simulink model "Parallel_n49"  (R2012b)
settings: Solver=VariableStepDiscrete  StartTime=0.0  StopTime=TotalIterations  RelTol=1e-3
values from neighbouring files (symbols this model uses):
  bp = 12    [ConfigValidate.m]
  bpSNMemory = bp    (= 12)    [ConfigValidate.m]
  IterationsOrdering = 4000    [ConfigValidate.m]
  MaxCoordDistance = (abs(max(wx) - min(wx))+abs(max(wy) - min(wy)))^2    [ConfigValidate.m]
  N_limit = 0.01    [ConfigValidate.m]
  nBits = 9    [ConfigValidate.m]
  nBitsNSmemories = (ceil(log2(TotalIterations)))    [ConfigValidate.m]
  S_limit = 1    [ConfigValidate.m]
  SourceNodes = 2000    [ConfigValidate.m]
  ts = 1    [ConfigValidate.m]
  w1 = rand(1,Neurons)    [ConfigValidate.m]
  w2 = rand(1,Neurons)    [ConfigValidate.m]
  wx = zeros(1,Neurons)    [ConfigValidate.m]
  wy = zeros(1,Neurons)    [ConfigValidate.m]
  x1 = rand(SourceNodes,1)    [ConfigValidate.m]
  x2 = rand(SourceNodes,1)    [ConfigValidate.m]
libraries: xbsIndex_r4 x4147, dspsrcs4 x2, dspstat3 x2
(part 3 of 19)

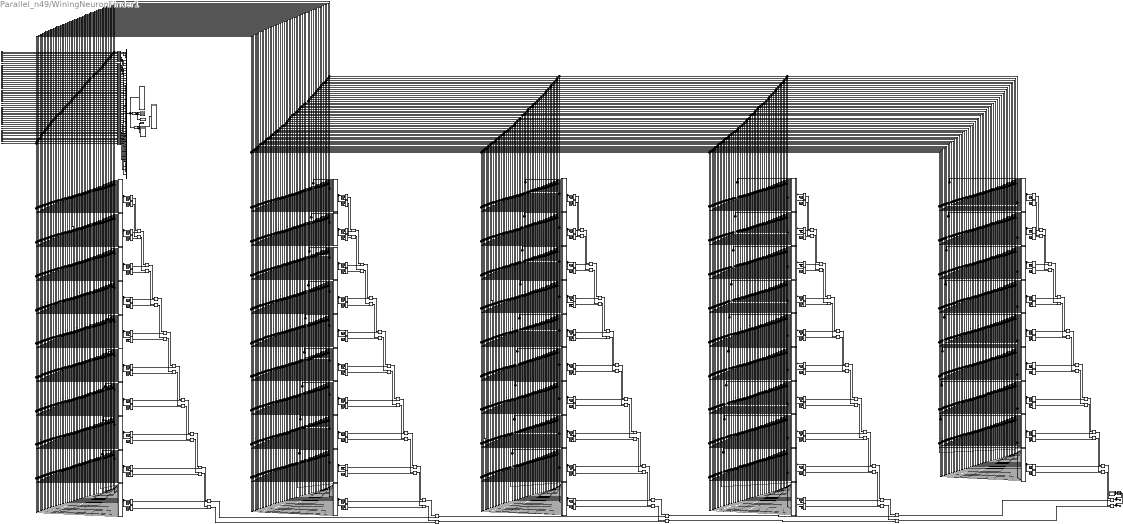
== system Parallel_n49/WiningNeuronFinder1 ==
  dist_k1 : Inport
  dist_k2 : Inport  Port=2
  dist_k3 : Inport  Port=3
  dist_k4 : Inport  Port=4
  dist_k5 : Inport  Port=5
  dist_k6 : Inport  Port=6
  dist_k7 : Inport  Port=7
  dist_k8 : Inport  Port=8
  dist_k9 : Inport  Port=9
  dist_k10 : Inport  Port=10
  dist_k11 : Inport  Port=11
  dist_k12 : Inport  Port=12
  dist_k13 : Inport  Port=13
  dist_k14 : Inport  Port=14
  dist_k15 : Inport  Port=15
  dist_k16 : Inport  Port=16
  dist_k17 : Inport  Port=17
  dist_k18 : Inport  Port=18
  dist_k19 : Inport  Port=19
  dist_k20 : Inport  Port=20
  dist_k21 : Inport  Port=21
  dist_k22 : Inport  Port=22
  dist_k23 : Inport  Port=23
  dist_k24 : Inport  Port=24
  dist_k25 : Inport  Port=25
  dist_k26 : Inport  Port=26
  dist_k27 : Inport  Port=27
  dist_k28 : Inport  Port=28
  dist_k29 : Inport  Port=29
  dist_k30 : Inport  Port=30
  dist_k31 : Inport  Port=31
  dist_k32 : Inport  Port=32
  dist_k33 : Inport  Port=33
  dist_k34 : Inport  Port=34
  dist_k35 : Inport  Port=35
  dist_k36 : Inport  Port=36
  dist_k37 : Inport  Port=37
  dist_k38 : Inport  Port=38
  dist_k39 : Inport  Port=39
  dist_k40 : Inport  Port=40
  dist_k41 : Inport  Port=41
  dist_k42 : Inport  Port=42
  dist_k43 : Inport  Port=43
  dist_k44 : Inport  Port=44
  dist_k45 : Inport  Port=45
  dist_k46 : Inport  Port=46
  dist_k47 : Inport  Port=47
  dist_k48 : Inport  Port=48
  dist_k49 : Inport  Port=49
  wx_1 : Inport  Port=50
  wy_1 : Inport  Port=51
  wx_2 : Inport  Port=52
  wy_2 : Inport  Port=53
  wx_3 : Inport  Port=54
  wy_3 : Inport  Port=55
  wx_4 : Inport  Port=56
  wy_4 : Inport  Port=57
  wx_5 : Inport  Port=58
  wy_5 : Inport  Port=59
  wx_6 : Inport  Port=60
  wy_6 : Inport  Port=61
  wx_7 : Inport  Port=62
  wy_7 : Inport  Port=63
  wx_8 : Inport  Port=64
  wy_8 : Inport  Port=65
  wx_9 : Inport  Port=66
  wy_9 : Inport  Port=67
  wx_10 : Inport  Port=68
  wy_10 : Inport  Port=69
  wx_11 : Inport  Port=70
  wy_11 : Inport  Port=71
  wx_12 : Inport  Port=72
  wy_12 : Inport  Port=73
  wx_13 : Inport  Port=74
  wy_13 : Inport  Port=75
  wx_14 : Inport  Port=76
  wy_14 : Inport  Port=77
  wx_15 : Inport  Port=78
  wy_15 : Inport  Port=79
  wx_16 : Inport  Port=80
  wy_16 : Inport  Port=81
  wx_17 : Inport  Port=82
  wy_17 : Inport  Port=83
  wx_18 : Inport  Port=84
  wy_18 : Inport  Port=85
  wx_19 : Inport  Port=86
  wy_19 : Inport  Port=87
  wx_20 : Inport  Port=88
  wy_20 : Inport  Port=89
  wx_21 : Inport  Port=90
  wy_21 : Inport  Port=91
  wx_22 : Inport  Port=92
  wy_22 : Inport  Port=93
  wx_23 : Inport  Port=94
  wy_23 : Inport  Port=95
  wx_24 : Inport  Port=96
  wy_24 : Inport  Port=97
  wx_25 : Inport  Port=98
  wy_25 : Inport  Port=99
  wx_26 : Inport  Port=100
  wy_26 : Inport  Port=101
  wx_27 : Inport  Port=102
  wy_27 : Inport  Port=103
  wx_28 : Inport  Port=104
  wy_28 : Inport  Port=105
  wx_29 : Inport  Port=106
  wy_29 : Inport  Port=107
  wx_30 : Inport  Port=108
  wy_30 : Inport  Port=109
  wx_31 : Inport  Port=110
  wy_31 : Inport  Port=111
  wx_32 : Inport  Port=112
  wy_32 : Inport  Port=113
  wx_33 : Inport  Port=114
  wy_33 : Inport  Port=115
  wx_34 : Inport  Port=116
  wy_34 : Inport  Port=117
  wx_35 : Inport  Port=118
  wy_35 : Inport  Port=119
  wx_36 : Inport  Port=120
  wy_36 : Inport  Port=121
  wx_37 : Inport  Port=122
  wy_37 : Inport  Port=123
  wx_38 : Inport  Port=124
  wy_38 : Inport  Port=125
  wx_39 : Inport  Port=126
  wy_39 : Inport  Port=127
  wx_40 : Inport  Port=128
  wy_40 : Inport  Port=129
  wx_41 : Inport  Port=130
  wy_41 : Inport  Port=131
  wx_42 : Inport  Port=132
  wy_42 : Inport  Port=133
  wx_43 : Inport  Port=134
  wy_43 : Inport  Port=135
  wx_44 : Inport  Port=136
  wy_44 : Inport  Port=137
  wx_45 : Inport  Port=138
  wy_45 : Inport  Port=139
  wx_46 : Inport  Port=140
  wy_46 : Inport  Port=141
  wx_47 : Inport  Port=142
  wy_47 : Inport  Port=143
  wx_48 : Inport  Port=144
  wy_48 : Inport  Port=145
  wx_49 : Inport  Port=146
  wy_49 : Inport  Port=147
  Display{,1..3,54..55} (6 alike) : Display
  Gateway Out{,1..28,31..42,44..53} (51 alike) : xbsIndex_r4/Gateway Out  inherit_from_input=off  hdl_port=off  timing_constraint=None  locs_specified=off  LOCs={}  UseAsDAC=off  DACChannel='1'  block_type=gatewayout
  LowerDist_n1 : Subsystem
  LowerDist_n10 : Subsystem
  LowerDist_n11 : Subsystem
  LowerDist_n12 : Subsystem
  LowerDist_n13 : Subsystem
  LowerDist_n14 : Subsystem
  LowerDist_n15 : Subsystem
  LowerDist_n16 : Subsystem
  LowerDist_n17 : Subsystem
  LowerDist_n18 : Subsystem
  LowerDist_n19 : Subsystem
  LowerDist_n2 : Subsystem
  LowerDist_n20 : Subsystem
  LowerDist_n21 : Subsystem
  LowerDist_n22 : Subsystem
  LowerDist_n23 : Subsystem
  LowerDist_n24 : Subsystem
  LowerDist_n25 : Subsystem
  LowerDist_n26 : Subsystem
  LowerDist_n27 : Subsystem
  LowerDist_n28 : Subsystem
  LowerDist_n29 : Subsystem
  LowerDist_n3 : Subsystem
  LowerDist_n30 : Subsystem
  LowerDist_n31 : Subsystem
  LowerDist_n32 : Subsystem
  LowerDist_n33 : Subsystem
  LowerDist_n34 : Subsystem
  LowerDist_n35 : Subsystem
  LowerDist_n36 : Subsystem
  LowerDist_n37 : Subsystem
  LowerDist_n38 : Subsystem
  LowerDist_n39 : Subsystem
  LowerDist_n4 : Subsystem
  LowerDist_n40 : Subsystem
  LowerDist_n41 : Subsystem
  LowerDist_n42 : Subsystem
  LowerDist_n43 : Subsystem
  LowerDist_n44 : Subsystem
  LowerDist_n45 : Subsystem
  LowerDist_n46 : Subsystem
  LowerDist_n47 : Subsystem
  LowerDist_n48 : Subsystem
  LowerDist_n49 : Subsystem
  LowerDist_n5 : Subsystem
  LowerDist_n6 : Subsystem
  LowerDist_n7 : Subsystem
  LowerDist_n8 : Subsystem
  LowerDist_n9 : Subsystem
  Minimum : dspstat3/Minimum  fcn=Value and Index  reset=None  InputProcessing=Columns as channels (frame based)  indexBase=One  operateOver=Each column  Dimension=1  colComp=on  operation=minimum  roiEnable=off  roiType=Rectangles  roiPortion=Entire ROI  roiOutput=Individual statistics for each ROI  roiFlag=off  roundingMode=Floor  overflowMode=off
  Mux : Mux  Inputs=49
  Mux2 : Mux  Inputs=2
  Sort : dspstat3/Sort  otype=Value and Index  dir=Ascending  sortAlg=Quick sort  accumDataTypeStr=Inherit: Same as product output  accumLastDataTypeStr=Inherit: Same as product output  roundingMode=Floor  overflowMode=off
  Sum_wxWinning_n{1..96} (96 alike) : xbsIndex_r4/AddSub  mode=Addition  use_carryin=off  use_carryout=off  en=off  latency=dAdd_CooperatingProcess  precision=User Defined  arith_type=Unsigned  n_bits=nbCoord  bin_pt=bpCoord  quantization=Truncate  overflow=Wrap  dbl_ovrd=off  use_behavioral_HDL=off  hw_selection=Fabric  pipelined=off  block_type=addsub
  To Workspace : ToWorkspace  VariableName=win_histH  SampleTime=ts
  To Workspace1 : ToWorkspace  VariableName=win_distH  SampleTime=ts
  wy_doMenor{,1..89,92..99} (98 alike) : xbsIndex_r4/Mux  inputs=2  en=off  latency=dMUX_CompetitiveProcess  precision=Full  arith_type=Unsigned  n_bits=16  bin_pt=14  quantization=Truncate  overflow=Wrap  dbl_ovrd=off  block_type=mux
  zero{,1..89,92..99} (98 alike) : xbsIndex_r4/Constant  const=0  gui_display_data_type=Fixed-point  arith_type=Unsigned  n_bits=nbCoord  bin_pt=bpCoord  preci_type=Single  exp_width=8  frac_width=24  explicit_period=on  period=ts  equ=P=C  opselect=C  inp2=PCIN>>17  opr=+  inp1=P  carry=CIN  dbl_ovrd=off  block_type=constant
  WinningNeuron_wx : Outport
  WinningNeuron_wy : Outport  Port=2
  wires:
  wy_1/1 -> wy_doMenor1/3
  wx_1/1 -> wy_doMenor/3
  Gateway Out6/1 -> Mux/7
  Gateway Out5/1 -> Mux/6
  Gateway Out7/1 -> Mux/8
  Gateway Out4/1 -> Mux/5
  Gateway Out8/1 -> Mux/9
  Gateway Out1/1 -> Mux/2
  Gateway Out3/1 -> Mux/4
  Gateway Out2/1 -> Mux/3
  Gateway Out10/1 -> Mux/11
  Gateway Out11/1 -> Mux/12
  Gateway Out9/1 -> Mux/10
  Gateway Out/1 -> Mux/1
  Gateway Out12/1 -> Mux/13
  Gateway Out22/1 -> Mux/17
  Gateway Out13/1 -> Mux/14
  Gateway Out14/1 -> Mux/15
  Gateway Out15/1 -> Mux/16
  Gateway Out23/1 -> Mux/18
  Gateway Out16/1 -> Mux/20
  Gateway Out17/1 -> Mux/21
  Gateway Out24/1 -> Mux/19
  Gateway Out18/1 -> Mux/22
  Gateway Out20/1 -> Mux/24
  Gateway Out21/1 -> Mux/25
  Gateway Out19/1 -> Mux/23
  LowerDist_n1/1(Out1) -> wy_doMenor1/1, wy_doMenor/1
  zero/1 -> wy_doMenor/2
  zero1/1 -> wy_doMenor1/2
  wy_doMenor/1 -> Sum_wxWinning_n1/1
  wy_doMenor1/1 -> Sum_wxWinning_n2/1
  Gateway Out25/1 -> Mux/26
  Gateway Out26/1 -> Mux/27
  Gateway Out41/1 -> Mux/28
  Gateway Out47/1 -> Mux/29
  Gateway Out48/1 -> Mux/30
  Gateway Out49/1 -> Mux/31
  Gateway Out51/1 -> Mux/33
  Gateway Out50/1 -> Mux/32
  Gateway Out52/1 -> Mux/34
  Gateway Out31/1 -> Mux/36
  Gateway Out32/1 -> Mux/37
  Gateway Out53/1 -> Mux/35
  Gateway Out33/1 -> Mux/38
  Gateway Out34/1 -> Mux/39
  Gateway Out35/1 -> Mux/40
  Gateway Out36/1 -> Mux/41
  Gateway Out44/1 -> Mux/42
  Gateway Out45/1 -> Mux/43
  Gateway Out38/1 -> Mux/46
  Gateway Out37/1 -> Mux/45
  Gateway Out46/1 -> Mux/44
  Gateway Out39/1 -> Mux/47
  Gateway Out42/1 -> Mux/49
  Gateway Out40/1 -> Mux/48
  wy_2/1 -> wy_doMenor3/3
  wx_2/1 -> wy_doMenor2/3
  LowerDist_n2/1(Out1) -> wy_doMenor3/1, wy_doMenor2/1
  zero2/1 -> wy_doMenor2/2
  zero3/1 -> wy_doMenor3/2
  wy_3/1 -> wy_doMenor5/3
  wx_3/1 -> wy_doMenor4/3
  LowerDist_n3/1(Out1) -> wy_doMenor5/1, wy_doMenor4/1
  zero4/1 -> wy_doMenor4/2
  zero5/1 -> wy_doMenor5/2
  wy_4/1 -> wy_doMenor7/3
  wx_4/1 -> wy_doMenor6/3
  LowerDist_n4/1(Out1) -> wy_doMenor7/1, wy_doMenor6/1
  zero6/1 -> wy_doMenor6/2
  zero7/1 -> wy_doMenor7/2
  wy_5/1 -> wy_doMenor9/3
  wx_5/1 -> wy_doMenor8/3
  LowerDist_n5/1(Out1) -> wy_doMenor9/1, wy_doMenor8/1
  zero8/1 -> wy_doMenor8/2
  zero9/1 -> wy_doMenor9/2
  wy_6/1 -> wy_doMenor11/3
  wx_6/1 -> wy_doMenor10/3
  LowerDist_n6/1(Out1) -> wy_doMenor11/1, wy_doMenor10/1
  zero10/1 -> wy_doMenor10/2
  zero11/1 -> wy_doMenor11/2
  wy_7/1 -> wy_doMenor13/3
  wx_7/1 -> wy_doMenor12/3
  LowerDist_n7/1(Out1) -> wy_doMenor13/1, wy_doMenor12/1
  zero12/1 -> wy_doMenor12/2
  zero13/1 -> wy_doMenor13/2
  wy_8/1 -> wy_doMenor15/3
  wx_8/1 -> wy_doMenor14/3
  LowerDist_n8/1(Out1) -> wy_doMenor15/1, wy_doMenor14/1
  zero14/1 -> wy_doMenor14/2
  zero15/1 -> wy_doMenor15/2
  wy_9/1 -> wy_doMenor17/3
  wx_9/1 -> wy_doMenor16/3
  LowerDist_n9/1(Out1) -> wy_doMenor17/1, wy_doMenor16/1
  zero16/1 -> wy_doMenor16/2
  zero17/1 -> wy_doMenor17/2
  wy_10/1 -> wy_doMenor19/3
  wx_10/1 -> wy_doMenor18/3
  LowerDist_n10/1(Out1) -> wy_doMenor19/1, wy_doMenor18/1
  zero18/1 -> wy_doMenor18/2
  zero19/1 -> wy_doMenor19/2
  wy_doMenor2/1 -> Sum_wxWinning_n1/2
  wy_doMenor3/1 -> Sum_wxWinning_n2/2
  Sum_wxWinning_n1/1 -> Sum_wxWinning_n3/1
  Sum_wxWinning_n2/1 -> Sum_wxWinning_n4/1
  wy_doMenor4/1 -> Sum_wxWinning_n3/2
  wy_doMenor5/1 -> Sum_wxWinning_n4/2
  Sum_wxWinning_n3/1 -> Sum_wxWinning_n5/1
  Sum_wxWinning_n4/1 -> Sum_wxWinning_n6/1
  wy_doMenor6/1 -> Sum_wxWinning_n5/2
  wy_doMenor7/1 -> Sum_wxWinning_n6/2
  Sum_wxWinning_n5/1 -> Sum_wxWinning_n7/1
  Sum_wxWinning_n6/1 -> Sum_wxWinning_n8/1
  wy_doMenor8/1 -> Sum_wxWinning_n7/2
  wy_doMenor9/1 -> Sum_wxWinning_n8/2
  Sum_wxWinning_n7/1 -> Sum_wxWinning_n9/1
  Sum_wxWinning_n8/1 -> Sum_wxWinning_n10/1
  wy_doMenor10/1 -> Sum_wxWinning_n9/2
  wy_doMenor11/1 -> Sum_wxWinning_n10/2
  Sum_wxWinning_n9/1 -> Sum_wxWinning_n11/1
  Sum_wxWinning_n10/1 -> Sum_wxWinning_n12/1
  wy_doMenor12/1 -> Sum_wxWinning_n11/2
  wy_doMenor13/1 -> Sum_wxWinning_n12/2
  Sum_wxWinning_n11/1 -> Sum_wxWinning_n13/1
  Sum_wxWinning_n12/1 -> Sum_wxWinning_n14/1
  wy_doMenor14/1 -> Sum_wxWinning_n13/2
  wy_doMenor15/1 -> Sum_wxWinning_n14/2
  Sum_wxWinning_n13/1 -> Sum_wxWinning_n15/1
  Sum_wxWinning_n14/1 -> Sum_wxWinning_n16/1
  wy_doMenor16/1 -> Sum_wxWinning_n15/2
  wy_doMenor17/1 -> Sum_wxWinning_n16/2
  Sum_wxWinning_n15/1 -> Sum_wxWinning_n17/1
  Sum_wxWinning_n16/1 -> Sum_wxWinning_n18/1
  wy_doMenor18/1 -> Sum_wxWinning_n17/2
  wy_doMenor19/1 -> Sum_wxWinning_n18/2
  wy_11/1 -> wy_doMenor21/3
  wx_11/1 -> wy_doMenor20/3
  LowerDist_n11/1(Out1) -> wy_doMenor21/1, wy_doMenor20/1
  zero20/1 -> wy_doMenor20/2
  zero21/1 -> wy_doMenor21/2
  wy_doMenor20/1 -> Sum_wxWinning_n19/1
  wy_doMenor21/1 -> Sum_wxWinning_n29/1
  wy_12/1 -> wy_doMenor33/3
  wx_12/1 -> wy_doMenor32/3
  LowerDist_n12/1(Out1) -> wy_doMenor33/1, wy_doMenor32/1
  zero32/1 -> wy_doMenor32/2
  zero33/1 -> wy_doMenor33/2
  wy_13/1 -> wy_doMenor35/3
  wx_13/1 -> wy_doMenor34/3
  LowerDist_n13/1(Out1) -> wy_doMenor35/1, wy_doMenor34/1
  zero34/1 -> wy_doMenor34/2
  zero35/1 -> wy_doMenor35/2
  wy_14/1 -> wy_doMenor37/3
  wx_14/1 -> wy_doMenor36/3
  LowerDist_n14/1(Out1) -> wy_doMenor37/1, wy_doMenor36/1
  zero36/1 -> wy_doMenor36/2
  zero37/1 -> wy_doMenor37/2
  wy_15/1 -> wy_doMenor39/3
  wx_15/1 -> wy_doMenor38/3
  LowerDist_n15/1(Out1) -> wy_doMenor39/1, wy_doMenor38/1
  zero38/1 -> wy_doMenor38/2
  zero39/1 -> wy_doMenor39/2
  wy_16/1 -> wy_doMenor23/3
  wx_16/1 -> wy_doMenor22/3
  LowerDist_n16/1(Out1) -> wy_doMenor23/1, wy_doMenor22/1
  zero22/1 -> wy_doMenor22/2
  zero23/1 -> wy_doMenor23/2
  wy_17/1 -> wy_doMenor25/3
  wx_17/1 -> wy_doMenor24/3
  LowerDist_n17/1(Out1) -> wy_doMenor25/1, wy_doMenor24/1
  zero24/1 -> wy_doMenor24/2
  zero25/1 -> wy_doMenor25/2
  wy_18/1 -> wy_doMenor27/3
  wx_18/1 -> wy_doMenor26/3
  LowerDist_n18/1(Out1) -> wy_doMenor27/1, wy_doMenor26/1
  zero26/1 -> wy_doMenor26/2
  zero27/1 -> wy_doMenor27/2
  wy_19/1 -> wy_doMenor29/3
  wx_19/1 -> wy_doMenor28/3
  LowerDist_n19/1(Out1) -> wy_doMenor29/1, wy_doMenor28/1
  zero28/1 -> wy_doMenor28/2
  zero29/1 -> wy_doMenor29/2
  wy_20/1 -> wy_doMenor31/3
  wx_20/1 -> wy_doMenor30/3
  LowerDist_n20/1(Out1) -> wy_doMenor31/1, wy_doMenor30/1
  zero30/1 -> wy_doMenor30/2
  zero31/1 -> wy_doMenor31/2
  wy_doMenor32/1 -> Sum_wxWinning_n19/2
  wy_doMenor33/1 -> Sum_wxWinning_n29/2
  Sum_wxWinning_n19/1 -> Sum_wxWinning_n30/1
  Sum_wxWinning_n29/1 -> Sum_wxWinning_n31/1
  wy_doMenor34/1 -> Sum_wxWinning_n30/2
  wy_doMenor35/1 -> Sum_wxWinning_n31/2
  Sum_wxWinning_n30/1 -> Sum_wxWinning_n32/1
  Sum_wxWinning_n31/1 -> Sum_wxWinning_n33/1
  wy_doMenor36/1 -> Sum_wxWinning_n32/2
  wy_doMenor37/1 -> Sum_wxWinning_n33/2
  Sum_wxWinning_n32/1 -> Sum_wxWinning_n34/1
  Sum_wxWinning_n33/1 -> Sum_wxWinning_n35/1
  wy_doMenor38/1 -> Sum_wxWinning_n34/2
  wy_doMenor39/1 -> Sum_wxWinning_n35/2
  Sum_wxWinning_n34/1 -> Sum_wxWinning_n36/1
  Sum_wxWinning_n35/1 -> Sum_wxWinning_n20/1
  wy_doMenor22/1 -> Sum_wxWinning_n36/2
  wy_doMenor23/1 -> Sum_wxWinning_n20/2
  Sum_wxWinning_n36/1 -> Sum_wxWinning_n21/1
  Sum_wxWinning_n20/1 -> Sum_wxWinning_n22/1
  wy_doMenor24/1 -> Sum_wxWinning_n21/2
  wy_doMenor25/1 -> Sum_wxWinning_n22/2
  Sum_wxWinning_n21/1 -> Sum_wxWinning_n23/1
  Sum_wxWinning_n22/1 -> Sum_wxWinning_n24/1
  wy_doMenor26/1 -> Sum_wxWinning_n23/2
  wy_doMenor27/1 -> Sum_wxWinning_n24/2
  Sum_wxWinning_n23/1 -> Sum_wxWinning_n25/1
  Sum_wxWinning_n24/1 -> Sum_wxWinning_n26/1
  wy_doMenor28/1 -> Sum_wxWinning_n25/2
  wy_doMenor29/1 -> Sum_wxWinning_n26/2
  Sum_wxWinning_n25/1 -> Sum_wxWinning_n27/1
  Sum_wxWinning_n26/1 -> Sum_wxWinning_n28/1
  wy_doMenor30/1 -> Sum_wxWinning_n27/2
  wy_doMenor31/1 -> Sum_wxWinning_n28/2
  Sum_wxWinning_n27/1 -> Sum_wxWinning_n37/1
  Sum_wxWinning_n17/1 -> Sum_wxWinning_n37/2
  Sum_wxWinning_n28/1 -> Sum_wxWinning_n38/1
  Sum_wxWinning_n18/1 -> Sum_wxWinning_n38/2
  wy_21/1 -> wy_doMenor41/3
  wx_21/1 -> wy_doMenor40/3
  LowerDist_n21/1(Out1) -> wy_doMenor41/1, wy_doMenor40/1
  zero40/1 -> wy_doMenor40/2
  zero41/1 -> wy_doMenor41/2
  wy_doMenor40/1 -> Sum_wxWinning_n39/1
  wy_doMenor41/1 -> Sum_wxWinning_n49/1
  wy_22/1 -> wy_doMenor53/3
  wx_22/1 -> wy_doMenor52/3
  LowerDist_n22/1(Out1) -> wy_doMenor53/1, wy_doMenor52/1
  zero52/1 -> wy_doMenor52/2
  zero53/1 -> wy_doMenor53/2
  wy_23/1 -> wy_doMenor55/3
  wx_23/1 -> wy_doMenor54/3
  LowerDist_n23/1(Out1) -> wy_doMenor55/1, wy_doMenor54/1
  zero54/1 -> wy_doMenor54/2
  zero55/1 -> wy_doMenor55/2
  wy_24/1 -> wy_doMenor57/3
  wx_24/1 -> wy_doMenor56/3
  LowerDist_n24/1(Out1) -> wy_doMenor57/1, wy_doMenor56/1
  zero56/1 -> wy_doMenor56/2
  zero57/1 -> wy_doMenor57/2
  wy_25/1 -> wy_doMenor59/3
  wx_25/1 -> wy_doMenor58/3
  LowerDist_n25/1(Out1) -> wy_doMenor59/1, wy_doMenor58/1
  zero58/1 -> wy_doMenor58/2
  zero59/1 -> wy_doMenor59/2
  wy_26/1 -> wy_doMenor43/3
  wx_26/1 -> wy_doMenor42/3
  LowerDist_n26/1(Out1) -> wy_doMenor43/1, wy_doMenor42/1
  zero42/1 -> wy_doMenor42/2
  zero43/1 -> wy_doMenor43/2
  wy_27/1 -> wy_doMenor45/3
  wx_27/1 -> wy_doMenor44/3
  LowerDist_n27/1(Out1) -> wy_doMenor45/1, wy_doMenor44/1
  zero44/1 -> wy_doMenor44/2
  zero45/1 -> wy_doMenor45/2
  wy_28/1 -> wy_doMenor47/3
  wx_28/1 -> wy_doMenor46/3
  LowerDist_n28/1(Out1) -> wy_doMenor47/1, wy_doMenor46/1
  zero46/1 -> wy_doMenor46/2
  zero47/1 -> wy_doMenor47/2
  wy_29/1 -> wy_doMenor49/3
  wx_29/1 -> wy_doMenor48/3
  LowerDist_n29/1(Out1) -> wy_doMenor49/1, wy_doMenor48/1
  zero48/1 -> wy_doMenor48/2
  zero49/1 -> wy_doMenor49/2
  wy_30/1 -> wy_doMenor51/3
  wx_30/1 -> wy_doMenor50/3
  LowerDist_n30/1(Out1) -> wy_doMenor51/1, wy_doMenor50/1
  zero50/1 -> wy_doMenor50/2
  zero51/1 -> wy_doMenor51/2
  wy_doMenor52/1 -> Sum_wxWinning_n39/2
  wy_doMenor53/1 -> Sum_wxWinning_n49/2
  Sum_wxWinning_n39/1 -> Sum_wxWinning_n50/1
  Sum_wxWinning_n49/1 -> Sum_wxWinning_n51/1
  wy_doMenor54/1 -> Sum_wxWinning_n50/2
  wy_doMenor55/1 -> Sum_wxWinning_n51/2
  Sum_wxWinning_n50/1 -> Sum_wxWinning_n52/1
  Sum_wxWinning_n51/1 -> Sum_wxWinning_n53/1
  wy_doMenor56/1 -> Sum_wxWinning_n52/2
  wy_doMenor57/1 -> Sum_wxWinning_n53/2
  Sum_wxWinning_n52/1 -> Sum_wxWinning_n54/1
  Sum_wxWinning_n53/1 -> Sum_wxWinning_n55/1
  wy_doMenor58/1 -> Sum_wxWinning_n54/2
  wy_doMenor59/1 -> Sum_wxWinning_n55/2
  Sum_wxWinning_n54/1 -> Sum_wxWinning_n56/1
  Sum_wxWinning_n55/1 -> Sum_wxWinning_n40/1
  wy_doMenor42/1 -> Sum_wxWinning_n56/2
  wy_doMenor43/1 -> Sum_wxWinning_n40/2
  Sum_wxWinning_n56/1 -> Sum_wxWinning_n41/1
  Sum_wxWinning_n40/1 -> Sum_wxWinning_n42/1
  wy_doMenor44/1 -> Sum_wxWinning_n41/2
  wy_doMenor45/1 -> Sum_wxWinning_n42/2
  Sum_wxWinning_n41/1 -> Sum_wxWinning_n43/1
  Sum_wxWinning_n42/1 -> Sum_wxWinning_n44/1
  wy_doMenor46/1 -> Sum_wxWinning_n43/2
  wy_doMenor47/1 -> Sum_wxWinning_n44/2
  Sum_wxWinning_n43/1 -> Sum_wxWinning_n45/1
  Sum_wxWinning_n44/1 -> Sum_wxWinning_n46/1
  wy_doMenor48/1 -> Sum_wxWinning_n45/2
  wy_doMenor49/1 -> Sum_wxWinning_n46/2
  Sum_wxWinning_n45/1 -> Sum_wxWinning_n47/1
  Sum_wxWinning_n46/1 -> Sum_wxWinning_n48/1
  wy_doMenor50/1 -> Sum_wxWinning_n47/2
  wy_doMenor51/1 -> Sum_wxWinning_n48/2
  Sum_wxWinning_n47/1 -> Sum_wxWinning_n57/1
  Sum_wxWinning_n37/1 -> Sum_wxWinning_n57/2
  Sum_wxWinning_n48/1 -> Sum_wxWinning_n58/1
  Sum_wxWinning_n38/1 -> Sum_wxWinning_n58/2
  wy_31/1 -> wy_doMenor61/3
  wx_31/1 -> wy_doMenor60/3
  LowerDist_n31/1(Out1) -> wy_doMenor61/1, wy_doMenor60/1
  zero60/1 -> wy_doMenor60/2
  zero61/1 -> wy_doMenor61/2
  wy_doMenor60/1 -> Sum_wxWinning_n59/1
  wy_doMenor61/1 -> Sum_wxWinning_n69/1
  wy_32/1 -> wy_doMenor73/3
  wx_32/1 -> wy_doMenor72/3
  LowerDist_n32/1(Out1) -> wy_doMenor73/1, wy_doMenor72/1
  zero72/1 -> wy_doMenor72/2
  zero73/1 -> wy_doMenor73/2
  wy_33/1 -> wy_doMenor75/3
  wx_33/1 -> wy_doMenor74/3
  LowerDist_n33/1(Out1) -> wy_doMenor75/1, wy_doMenor74/1
  zero74/1 -> wy_doMenor74/2
  zero75/1 -> wy_doMenor75/2
  wy_34/1 -> wy_doMenor77/3
  wx_34/1 -> wy_doMenor76/3
  LowerDist_n34/1(Out1) -> wy_doMenor77/1, wy_doMenor76/1
  zero76/1 -> wy_doMenor76/2
  zero77/1 -> wy_doMenor77/2
  wy_35/1 -> wy_doMenor79/3
  wx_35/1 -> wy_doMenor78/3
  LowerDist_n35/1(Out1) -> wy_doMenor79/1, wy_doMenor78/1
  zero78/1 -> wy_doMenor78/2
  zero79/1 -> wy_doMenor79/2
  wy_36/1 -> wy_doMenor63/3
  wx_36/1 -> wy_doMenor62/3
  LowerDist_n36/1(Out1) -> wy_doMenor63/1, wy_doMenor62/1
  zero62/1 -> wy_doMenor62/2
  zero63/1 -> wy_doMenor63/2
  wy_37/1 -> wy_doMenor65/3
  wx_37/1 -> wy_doMenor64/3
  LowerDist_n37/1(Out1) -> wy_doMenor65/1, wy_doMenor64/1
  zero64/1 -> wy_doMenor64/2
  zero65/1 -> wy_doMenor65/2
  wy_38/1 -> wy_doMenor67/3
  wx_38/1 -> wy_doMenor66/3
  LowerDist_n38/1(Out1) -> wy_doMenor67/1, wy_doMenor66/1
  zero66/1 -> wy_doMenor66/2
  zero67/1 -> wy_doMenor67/2
  wy_39/1 -> wy_doMenor69/3
  wx_39/1 -> wy_doMenor68/3
  LowerDist_n39/1(Out1) -> wy_doMenor69/1, wy_doMenor68/1
  zero68/1 -> wy_doMenor68/2
  zero69/1 -> wy_doMenor69/2
  wy_40/1 -> wy_doMenor71/3
  wx_40/1 -> wy_doMenor70/3
  LowerDist_n40/1(Out1) -> wy_doMenor71/1, wy_doMenor70/1
  zero70/1 -> wy_doMenor70/2
  zero71/1 -> wy_doMenor71/2
  wy_doMenor72/1 -> Sum_wxWinning_n59/2
  wy_doMenor73/1 -> Sum_wxWinning_n69/2
  Sum_wxWinning_n59/1 -> Sum_wxWinning_n70/1
  Sum_wxWinning_n69/1 -> Sum_wxWinning_n71/1
  wy_doMenor74/1 -> Sum_wxWinning_n70/2
  wy_doMenor75/1 -> Sum_wxWinning_n71/2
  Sum_wxWinning_n70/1 -> Sum_wxWinning_n72/1
  Sum_wxWinning_n71/1 -> Sum_wxWinning_n73/1
  wy_doMenor76/1 -> Sum_wxWinning_n72/2
  wy_doMenor77/1 -> Sum_wxWinning_n73/2
  Sum_wxWinning_n72/1 -> Sum_wxWinning_n74/1
  Sum_wxWinning_n73/1 -> Sum_wxWinning_n75/1
  wy_doMenor78/1 -> Sum_wxWinning_n74/2
  wy_doMenor79/1 -> Sum_wxWinning_n75/2
  Sum_wxWinning_n74/1 -> Sum_wxWinning_n76/1
  Sum_wxWinning_n75/1 -> Sum_wxWinning_n60/1
  wy_doMenor62/1 -> Sum_wxWinning_n76/2
  wy_doMenor63/1 -> Sum_wxWinning_n60/2
  Sum_wxWinning_n76/1 -> Sum_wxWinning_n61/1
  Sum_wxWinning_n60/1 -> Sum_wxWinning_n62/1
  wy_doMenor64/1 -> Sum_wxWinning_n61/2
  wy_doMenor65/1 -> Sum_wxWinning_n62/2
  Sum_wxWinning_n61/1 -> Sum_wxWinning_n63/1
  Sum_wxWinning_n62/1 -> Sum_wxWinning_n64/1
  wy_doMenor66/1 -> Sum_wxWinning_n63/2
  wy_doMenor67/1 -> Sum_wxWinning_n64/2
  Sum_wxWinning_n63/1 -> Sum_wxWinning_n65/1
  Sum_wxWinning_n64/1 -> Sum_wxWinning_n66/1
  wy_doMenor68/1 -> Sum_wxWinning_n65/2
  wy_doMenor69/1 -> Sum_wxWinning_n66/2
  Sum_wxWinning_n65/1 -> Sum_wxWinning_n67/1
  Sum_wxWinning_n66/1 -> Sum_wxWinning_n68/1
  wy_doMenor70/1 -> Sum_wxWinning_n67/2
  wy_doMenor71/1 -> Sum_wxWinning_n68/2
  Sum_wxWinning_n67/1 -> Sum_wxWinning_n77/1
  Sum_wxWinning_n57/1 -> Sum_wxWinning_n77/2
  Sum_wxWinning_n68/1 -> Sum_wxWinning_n78/1
  Sum_wxWinning_n58/1 -> Sum_wxWinning_n78/2
  wy_41/1 -> wy_doMenor81/3
  wx_41/1 -> wy_doMenor80/3
  LowerDist_n41/1(Out1) -> wy_doMenor81/1, wy_doMenor80/1
  zero80/1 -> wy_doMenor80/2
  zero81/1 -> wy_doMenor81/2
  wy_doMenor80/1 -> Sum_wxWinning_n79/1
  wy_doMenor81/1 -> Sum_wxWinning_n89/1
  wy_42/1 -> wy_doMenor93/3
  wx_42/1 -> wy_doMenor92/3
  LowerDist_n42/1(Out1) -> wy_doMenor93/1, wy_doMenor92/1
  zero92/1 -> wy_doMenor92/2
  zero93/1 -> wy_doMenor93/2
  wy_43/1 -> wy_doMenor95/3
  wx_43/1 -> wy_doMenor94/3
  LowerDist_n43/1(Out1) -> wy_doMenor95/1, wy_doMenor94/1
  zero94/1 -> wy_doMenor94/2
  zero95/1 -> wy_doMenor95/2
  wy_44/1 -> wy_doMenor97/3
  wx_44/1 -> wy_doMenor96/3
  LowerDist_n44/1(Out1) -> wy_doMenor97/1, wy_doMenor96/1
  zero96/1 -> wy_doMenor96/2
  zero97/1 -> wy_doMenor97/2
  wy_45/1 -> wy_doMenor99/3
  wx_45/1 -> wy_doMenor98/3
  LowerDist_n45/1(Out1) -> wy_doMenor99/1, wy_doMenor98/1
  zero98/1 -> wy_doMenor98/2
  zero99/1 -> wy_doMenor99/2
  wy_46/1 -> wy_doMenor83/3
  wx_46/1 -> wy_doMenor82/3
  LowerDist_n46/1(Out1) -> wy_doMenor83/1, wy_doMenor82/1
  zero82/1 -> wy_doMenor82/2
  zero83/1 -> wy_doMenor83/2
  wy_47/1 -> wy_doMenor85/3
  wx_47/1 -> wy_doMenor84/3
  LowerDist_n47/1(Out1) -> wy_doMenor85/1, wy_doMenor84/1
  zero84/1 -> wy_doMenor84/2
  zero85/1 -> wy_doMenor85/2
  wy_48/1 -> wy_doMenor87/3
  wx_48/1 -> wy_doMenor86/3
  LowerDist_n48/1(Out1) -> wy_doMenor87/1, wy_doMenor86/1
  zero86/1 -> wy_doMenor86/2
  zero87/1 -> wy_doMenor87/2
  wy_49/1 -> wy_doMenor89/3
  wx_49/1 -> wy_doMenor88/3
  LowerDist_n49/1(Out1) -> wy_doMenor89/1, wy_doMenor88/1
  zero88/1 -> wy_doMenor88/2
  zero89/1 -> wy_doMenor89/2
  wy_doMenor92/1 -> Sum_wxWinning_n79/2
  wy_doMenor93/1 -> Sum_wxWinning_n89/2
  Sum_wxWinning_n79/1 -> Sum_wxWinning_n90/1
  Sum_wxWinning_n89/1 -> Sum_wxWinning_n91/1
  wy_doMenor94/1 -> Sum_wxWinning_n90/2
  wy_doMenor95/1 -> Sum_wxWinning_n91/2
  Sum_wxWinning_n90/1 -> Sum_wxWinning_n92/1
  Sum_wxWinning_n91/1 -> Sum_wxWinning_n93/1
  wy_doMenor96/1 -> Sum_wxWinning_n92/2
  wy_doMenor97/1 -> Sum_wxWinning_n93/2
  Sum_wxWinning_n92/1 -> Sum_wxWinning_n94/1
  Sum_wxWinning_n93/1 -> Sum_wxWinning_n95/1
  wy_doMenor98/1 -> Sum_wxWinning_n94/2
  wy_doMenor99/1 -> Sum_wxWinning_n95/2
  Sum_wxWinning_n94/1 -> Sum_wxWinning_n96/1
  Sum_wxWinning_n95/1 -> Sum_wxWinning_n80/1
  wy_doMenor82/1 -> Sum_wxWinning_n96/2
  wy_doMenor83/1 -> Sum_wxWinning_n80/2
  Sum_wxWinning_n96/1 -> Sum_wxWinning_n81/1
  Sum_wxWinning_n80/1 -> Sum_wxWinning_n82/1
  wy_doMenor84/1 -> Sum_wxWinning_n81/2
  wy_doMenor85/1 -> Sum_wxWinning_n82/2
  Sum_wxWinning_n81/1 -> Sum_wxWinning_n83/1
  Sum_wxWinning_n82/1 -> Sum_wxWinning_n84/1
  wy_doMenor86/1 -> Sum_wxWinning_n83/2
  wy_doMenor87/1 -> Sum_wxWinning_n84/2
  Sum_wxWinning_n83/1 -> Sum_wxWinning_n85/1
  Sum_wxWinning_n84/1 -> Sum_wxWinning_n86/1
  wy_doMenor88/1 -> Sum_wxWinning_n85/2
  wy_doMenor89/1 -> Sum_wxWinning_n86/2
  Sum_wxWinning_n85/1 -> Sum_wxWinning_n87/1
  Sum_wxWinning_n86/1 -> Sum_wxWinning_n88/1
  dist_k3/1 -> LowerDist_n42/3(In3), LowerDist_n43/3(In3), LowerDist_n47/3(In3), LowerDist_n49/3(In3), LowerDist_n48/3(In3), LowerDist_n46/3(In3), LowerDist_n45/3(In3), LowerDist_n44/3(In3), LowerDist_n41/3(In3), LowerDist_n31/3(In3), LowerDist_n32/3(In3), LowerDist_n33/3(In3), LowerDist_n37/3(In3), LowerDist_n40/3(In3), LowerDist_n39/3(In3), LowerDist_n38/3(In3), LowerDist_n36/3(In3), LowerDist_n35/3(In3), LowerDist_n34/3(In3), LowerDist_n22/3(In3), LowerDist_n23/3(In3), LowerDist_n27/3(In3), LowerDist_n30/3(In3), LowerDist_n29/3(In3), LowerDist_n28/3(In3), LowerDist_n26/3(In3), LowerDist_n25/3(In3), LowerDist_n24/3(In3), LowerDist_n21/3(In3), LowerDist_n12/3(In3), LowerDist_n13/3(In3), LowerDist_n17/3(In3), LowerDist_n20/3(In3), LowerDist_n19/3(In3), LowerDist_n18/3(In3), LowerDist_n16/3(In3), LowerDist_n15/3(In3), LowerDist_n14/3(In3), LowerDist_n11/3(In3), LowerDist_n3/1(In1), LowerDist_n7/3(In3), LowerDist_n10/3(In3), LowerDist_n9/3(In3), LowerDist_n8/3(In3), LowerDist_n6/3(In3), LowerDist_n5/3(In3), LowerDist_n4/3(In3), LowerDist_n2/3(In3), LowerDist_n1/3(In3), Gateway Out2/1
  dist_k25/1 -> LowerDist_n45/25(In25), LowerDist_n49/25(In25), LowerDist_n48/25(In25), LowerDist_n47/25(In25), LowerDist_n46/25(In25), LowerDist_n44/25(In25), LowerDist_n43/25(In25), LowerDist_n42/25(In25), LowerDist_n41/25(In25), LowerDist_n31/25(In25), LowerDist_n35/25(In25), LowerDist_n40/25(In25), LowerDist_n39/25(In25), LowerDist_n38/25(In25), LowerDist_n37/25(In25), LowerDist_n36/25(In25), LowerDist_n34/25(In25), LowerDist_n33/25(In25), LowerDist_n32/25(In25), LowerDist_n30/25(In25), LowerDist_n29/25(In25), LowerDist_n28/25(In25), LowerDist_n27/25(In25), LowerDist_n26/25(In25), LowerDist_n25/1(In1), LowerDist_n24/25(In25), LowerDist_n23/25(In25), LowerDist_n22/25(In25), LowerDist_n21/25(In25), LowerDist_n20/25(In25), LowerDist_n19/25(In25), LowerDist_n18/25(In25), LowerDist_n17/25(In25), LowerDist_n16/25(In25), LowerDist_n15/25(In25), LowerDist_n14/25(In25), LowerDist_n13/25(In25), LowerDist_n12/25(In25), LowerDist_n11/25(In25), LowerDist_n10/25(In25), LowerDist_n9/25(In25), LowerDist_n8/25(In25), LowerDist_n7/25(In25), LowerDist_n6/25(In25), LowerDist_n5/25(In25), LowerDist_n4/25(In25), LowerDist_n3/25(In25), LowerDist_n2/25(In25), LowerDist_n1/25(In25), Gateway Out21/1
  dist_k15/1 -> LowerDist_n10/15(In15), LowerDist_n9/15(In15), LowerDist_n8/15(In15), LowerDist_n7/15(In15), LowerDist_n6/15(In15), LowerDist_n5/15(In15), LowerDist_n4/15(In15), LowerDist_n3/15(In15), LowerDist_n2/15(In15), LowerDist_n1/15(In15), LowerDist_n45/15(In15), LowerDist_n49/15(In15), LowerDist_n48/15(In15), LowerDist_n47/15(In15), LowerDist_n46/15(In15), LowerDist_n44/15(In15), LowerDist_n43/15(In15), LowerDist_n42/15(In15), LowerDist_n41/15(In15), LowerDist_n31/15(In15), LowerDist_n35/15(In15), LowerDist_n40/15(In15), LowerDist_n39/15(In15), LowerDist_n38/15(In15), LowerDist_n37/15(In15), LowerDist_n36/15(In15), LowerDist_n34/15(In15), LowerDist_n33/15(In15), LowerDist_n32/15(In15), LowerDist_n25/15(In15), LowerDist_n30/15(In15), LowerDist_n29/15(In15), LowerDist_n28/15(In15), LowerDist_n27/15(In15), LowerDist_n26/15(In15), LowerDist_n24/15(In15), LowerDist_n23/15(In15), LowerDist_n22/15(In15), LowerDist_n21/15(In15), LowerDist_n20/15(In15), LowerDist_n19/15(In15), LowerDist_n18/15(In15), LowerDist_n17/15(In15), LowerDist_n16/15(In15), LowerDist_n15/1(In1), LowerDist_n14/15(In15), LowerDist_n13/15(In15), LowerDist_n12/15(In15), LowerDist_n11/15(In15), Gateway Out14/1
  dist_k4/1 -> LowerDist_n12/4(In4), LowerDist_n14/4(In4), LowerDist_n18/4(In4), LowerDist_n20/4(In4), LowerDist_n19/4(In4), LowerDist_n17/4(In4), LowerDist_n16/4(In4), LowerDist_n15/4(In4), LowerDist_n13/4(In4), LowerDist_n11/4(In4), LowerDist_n42/4(In4), LowerDist_n44/4(In4), LowerDist_n48/4(In4), LowerDist_n49/4(In4), LowerDist_n47/4(In4), LowerDist_n46/4(In4), LowerDist_n45/4(In4), LowerDist_n43/4(In4), LowerDist_n41/4(In4), LowerDist_n31/4(In4), LowerDist_n32/4(In4), LowerDist_n34/4(In4), LowerDist_n38/4(In4), LowerDist_n40/4(In4), LowerDist_n39/4(In4), LowerDist_n37/4(In4), LowerDist_n36/4(In4), LowerDist_n35/4(In4), LowerDist_n33/4(In4), LowerDist_n22/4(In4), LowerDist_n24/4(In4), LowerDist_n28/4(In4), LowerDist_n30/4(In4), LowerDist_n29/4(In4), LowerDist_n27/4(In4), LowerDist_n26/4(In4), LowerDist_n25/4(In4), LowerDist_n23/4(In4), LowerDist_n21/4(In4), LowerDist_n4/1(In1), LowerDist_n8/4(In4), LowerDist_n10/4(In4), LowerDist_n9/4(In4), LowerDist_n7/4(In4), LowerDist_n6/4(In4), LowerDist_n5/4(In4), LowerDist_n3/4(In4), LowerDist_n2/4(In4), LowerDist_n1/4(In4), Gateway Out3/1
  dist_k7/1 -> LowerDist_n12/7(In7), LowerDist_n17/7(In7), LowerDist_n19/7(In7), LowerDist_n20/7(In7), LowerDist_n18/7(In7), LowerDist_n16/7(In7), LowerDist_n15/7(In7), LowerDist_n14/7(In7), LowerDist_n13/7(In7), LowerDist_n11/7(In7), LowerDist_n22/7(In7), LowerDist_n27/7(In7), LowerDist_n29/7(In7), LowerDist_n30/7(In7), LowerDist_n28/7(In7), LowerDist_n26/7(In7), LowerDist_n25/7(In7), LowerDist_n24/7(In7), LowerDist_n23/7(In7), LowerDist_n21/7(In7), LowerDist_n42/7(In7), LowerDist_n47/7(In7), LowerDist_n49/7(In7), LowerDist_n48/7(In7), LowerDist_n46/7(In7), LowerDist_n45/7(In7), LowerDist_n44/7(In7), LowerDist_n43/7(In7), LowerDist_n41/7(In7), LowerDist_n31/7(In7), LowerDist_n32/7(In7), LowerDist_n37/7(In7), LowerDist_n39/7(In7), LowerDist_n40/7(In7), LowerDist_n38/7(In7), LowerDist_n36/7(In7), LowerDist_n35/7(In7), LowerDist_n34/7(In7), LowerDist_n33/7(In7), LowerDist_n9/7(In7), LowerDist_n10/7(In7), LowerDist_n8/7(In7), LowerDist_n7/1(In1), LowerDist_n6/7(In7), LowerDist_n5/7(In7), LowerDist_n4/7(In7), LowerDist_n3/7(In7), LowerDist_n2/7(In7), LowerDist_n1/7(In7), Gateway Out6/1
  dist_k9/1 -> LowerDist_n12/9(In9), LowerDist_n19/9(In9), LowerDist_n20/9(In9), LowerDist_n18/9(In9), LowerDist_n17/9(In9), LowerDist_n16/9(In9), LowerDist_n15/9(In9), LowerDist_n14/9(In9), LowerDist_n13/9(In9), LowerDist_n11/9(In9), LowerDist_n22/9(In9), LowerDist_n29/9(In9), LowerDist_n30/9(In9), LowerDist_n28/9(In9), LowerDist_n27/9(In9), LowerDist_n26/9(In9), LowerDist_n25/9(In9), LowerDist_n24/9(In9), LowerDist_n23/9(In9), LowerDist_n21/9(In9), LowerDist_n42/9(In9), LowerDist_n49/9(In9), LowerDist_n48/9(In9), LowerDist_n47/9(In9), LowerDist_n46/9(In9), LowerDist_n45/9(In9), LowerDist_n44/9(In9), LowerDist_n43/9(In9), LowerDist_n41/9(In9), LowerDist_n31/9(In9), LowerDist_n32/9(In9), LowerDist_n39/9(In9), LowerDist_n40/9(In9), LowerDist_n38/9(In9), LowerDist_n37/9(In9), LowerDist_n36/9(In9), LowerDist_n35/9(In9), LowerDist_n34/9(In9), LowerDist_n33/9(In9), LowerDist_n9/1(In1), LowerDist_n10/9(In9), LowerDist_n8/9(In9), LowerDist_n7/9(In9), LowerDist_n6/9(In9), LowerDist_n5/9(In9), LowerDist_n4/9(In9), LowerDist_n3/9(In9), LowerDist_n2/9(In9), LowerDist_n1/9(In9), Gateway Out8/1
  dist_k11/1 -> LowerDist_n10/11(In11), LowerDist_n9/11(In11), LowerDist_n8/11(In11), LowerDist_n7/11(In11), LowerDist_n6/11(In11), LowerDist_n5/11(In11), LowerDist_n4/11(In11), LowerDist_n3/11(In11), LowerDist_n2/11(In11), LowerDist_n1/11(In11), LowerDist_n11/1(In1), LowerDist_n12/11(In11), LowerDist_n20/11(In11), LowerDist_n19/11(In11), LowerDist_n18/11(In11), LowerDist_n17/11(In11), LowerDist_n16/11(In11), LowerDist_n15/11(In11), LowerDist_n14/11(In11), LowerDist_n13/11(In11), LowerDist_n21/11(In11), LowerDist_n22/11(In11), LowerDist_n30/11(In11), LowerDist_n29/11(In11), LowerDist_n28/11(In11), LowerDist_n27/11(In11), LowerDist_n26/11(In11), LowerDist_n25/11(In11), LowerDist_n24/11(In11), LowerDist_n23/11(In11), LowerDist_n41/11(In11), LowerDist_n42/11(In11), LowerDist_n49/11(In11), LowerDist_n48/11(In11), LowerDist_n47/11(In11), LowerDist_n46/11(In11), LowerDist_n45/11(In11), LowerDist_n44/11(In11), LowerDist_n43/11(In11), LowerDist_n31/11(In11), LowerDist_n32/11(In11), LowerDist_n40/11(In11), LowerDist_n39/11(In11), LowerDist_n38/11(In11), LowerDist_n37/11(In11), LowerDist_n36/11(In11), LowerDist_n35/11(In11), LowerDist_n34/11(In11), LowerDist_n33/11(In11), Gateway Out10/1
  dist_k13/1 -> LowerDist_n10/13(In13), LowerDist_n9/13(In13), LowerDist_n8/13(In13), LowerDist_n7/13(In13), LowerDist_n6/13(In13), LowerDist_n5/13(In13), LowerDist_n4/13(In13), LowerDist_n3/13(In13), LowerDist_n2/13(In13), LowerDist_n1/13(In13), LowerDist_n20/13(In13), LowerDist_n19/13(In13), LowerDist_n18/13(In13), LowerDist_n17/13(In13), LowerDist_n16/13(In13), LowerDist_n15/13(In13), LowerDist_n14/13(In13), LowerDist_n13/1(In1), LowerDist_n12/13(In13), LowerDist_n11/13(In13), LowerDist_n23/13(In13), LowerDist_n30/13(In13), LowerDist_n29/13(In13), LowerDist_n28/13(In13), LowerDist_n27/13(In13), LowerDist_n26/13(In13), LowerDist_n25/13(In13), LowerDist_n24/13(In13), LowerDist_n22/13(In13), LowerDist_n21/13(In13), LowerDist_n43/13(In13), LowerDist_n49/13(In13), LowerDist_n48/13(In13), LowerDist_n47/13(In13), LowerDist_n46/13(In13), LowerDist_n45/13(In13), LowerDist_n44/13(In13), LowerDist_n42/13(In13), LowerDist_n41/13(In13), LowerDist_n31/13(In13), LowerDist_n33/13(In13), LowerDist_n40/13(In13), LowerDist_n39/13(In13), LowerDist_n38/13(In13), LowerDist_n37/13(In13), LowerDist_n36/13(In13), LowerDist_n35/13(In13), LowerDist_n34/13(In13), LowerDist_n32/13(In13), Gateway Out12/1
  dist_k14/1 -> LowerDist_n10/14(In14), LowerDist_n9/14(In14), LowerDist_n8/14(In14), LowerDist_n7/14(In14), LowerDist_n6/14(In14), LowerDist_n5/14(In14), LowerDist_n4/14(In14), LowerDist_n3/14(In14), LowerDist_n2/14(In14), LowerDist_n1/14(In14), LowerDist_n44/14(In14), LowerDist_n49/14(In14), LowerDist_n48/14(In14), LowerDist_n47/14(In14), LowerDist_n46/14(In14), LowerDist_n45/14(In14), LowerDist_n43/14(In14), LowerDist_n42/14(In14), LowerDist_n41/14(In14), LowerDist_n31/14(In14), LowerDist_n34/14(In14), LowerDist_n40/14(In14), LowerDist_n39/14(In14), LowerDist_n38/14(In14), LowerDist_n37/14(In14), LowerDist_n36/14(In14), LowerDist_n35/14(In14), LowerDist_n33/14(In14), LowerDist_n32/14(In14), LowerDist_n24/14(In14), LowerDist_n30/14(In14), LowerDist_n29/14(In14), LowerDist_n28/14(In14), LowerDist_n27/14(In14), LowerDist_n26/14(In14), LowerDist_n25/14(In14), LowerDist_n23/14(In14), LowerDist_n22/14(In14), LowerDist_n21/14(In14), LowerDist_n20/14(In14), LowerDist_n19/14(In14), LowerDist_n18/14(In14), LowerDist_n17/14(In14), LowerDist_n16/14(In14), LowerDist_n15/14(In14), LowerDist_n14/1(In1), LowerDist_n13/14(In14), LowerDist_n12/14(In14), LowerDist_n11/14(In14), Gateway Out13/1
  dist_k17/1 -> LowerDist_n10/17(In17), LowerDist_n9/17(In17), LowerDist_n8/17(In17), LowerDist_n7/17(In17), LowerDist_n6/17(In17), LowerDist_n5/17(In17), LowerDist_n4/17(In17), LowerDist_n3/17(In17), LowerDist_n2/17(In17), LowerDist_n1/17(In17), LowerDist_n20/17(In17), LowerDist_n19/17(In17), LowerDist_n18/17(In17), LowerDist_n17/1(In1), LowerDist_n16/17(In17), LowerDist_n15/17(In17), LowerDist_n14/17(In17), LowerDist_n13/17(In17), LowerDist_n12/17(In17), LowerDist_n11/17(In17), LowerDist_n47/17(In17), LowerDist_n49/17(In17), LowerDist_n48/17(In17), LowerDist_n46/17(In17), LowerDist_n45/17(In17), LowerDist_n44/17(In17), LowerDist_n43/17(In17), LowerDist_n42/17(In17), LowerDist_n41/17(In17), LowerDist_n31/17(In17), LowerDist_n37/17(In17), LowerDist_n40/17(In17), LowerDist_n39/17(In17), LowerDist_n38/17(In17), LowerDist_n36/17(In17), LowerDist_n35/17(In17), LowerDist_n34/17(In17), LowerDist_n33/17(In17), LowerDist_n32/17(In17), LowerDist_n27/17(In17), LowerDist_n30/17(In17), LowerDist_n29/17(In17), LowerDist_n28/17(In17), LowerDist_n26/17(In17), LowerDist_n25/17(In17), LowerDist_n24/17(In17), LowerDist_n23/17(In17), LowerDist_n22/17(In17), LowerDist_n21/17(In17), Gateway Out22/1
  dist_k18/1 -> LowerDist_n4/18(In18), LowerDist_n10/18(In18), LowerDist_n9/18(In18), LowerDist_n8/18(In18), LowerDist_n7/18(In18), LowerDist_n6/18(In18), LowerDist_n5/18(In18), LowerDist_n3/18(In18), LowerDist_n2/18(In18), LowerDist_n1/18(In18), LowerDist_n14/18(In18), LowerDist_n20/18(In18), LowerDist_n19/18(In18), LowerDist_n18/1(In1), LowerDist_n17/18(In18), LowerDist_n16/18(In18), LowerDist_n15/18(In18), LowerDist_n13/18(In18), LowerDist_n12/18(In18), LowerDist_n11/18(In18), LowerDist_n44/18(In18), LowerDist_n48/18(In18), LowerDist_n49/18(In18), LowerDist_n47/18(In18), LowerDist_n46/18(In18), LowerDist_n45/18(In18), LowerDist_n43/18(In18), LowerDist_n42/18(In18), LowerDist_n41/18(In18), LowerDist_n31/18(In18), LowerDist_n34/18(In18), LowerDist_n38/18(In18), LowerDist_n40/18(In18), LowerDist_n39/18(In18), LowerDist_n37/18(In18), LowerDist_n36/18(In18), LowerDist_n35/18(In18), LowerDist_n33/18(In18), LowerDist_n32/18(In18), LowerDist_n24/18(In18), LowerDist_n28/18(In18), LowerDist_n30/18(In18), LowerDist_n29/18(In18), LowerDist_n27/18(In18), LowerDist_n26/18(In18), LowerDist_n25/18(In18), LowerDist_n23/18(In18), LowerDist_n22/18(In18), LowerDist_n21/18(In18), Gateway Out23/1
  dist_k19/1 -> LowerDist_n20/19(In19), LowerDist_n19/1(In1), LowerDist_n18/19(In19), LowerDist_n17/19(In19), LowerDist_n16/19(In19), LowerDist_n15/19(In19), LowerDist_n14/19(In19), LowerDist_n13/19(In19), LowerDist_n12/19(In19), LowerDist_n11/19(In19), LowerDist_n29/19(In19), LowerDist_n30/19(In19), LowerDist_n28/19(In19), LowerDist_n27/19(In19), LowerDist_n26/19(In19), LowerDist_n25/19(In19), LowerDist_n24/19(In19), LowerDist_n23/19(In19), LowerDist_n22/19(In19), LowerDist_n21/19(In19), LowerDist_n49/19(In19), LowerDist_n48/19(In19), LowerDist_n47/19(In19), LowerDist_n46/19(In19), LowerDist_n45/19(In19), LowerDist_n44/19(In19), LowerDist_n43/19(In19), LowerDist_n42/19(In19), LowerDist_n41/19(In19), LowerDist_n31/19(In19), LowerDist_n39/19(In19), LowerDist_n40/19(In19), LowerDist_n38/19(In19), LowerDist_n37/19(In19), LowerDist_n36/19(In19), LowerDist_n35/19(In19), LowerDist_n34/19(In19), LowerDist_n33/19(In19), LowerDist_n32/19(In19), LowerDist_n10/19(In19), LowerDist_n9/19(In19), LowerDist_n8/19(In19), LowerDist_n7/19(In19), LowerDist_n6/19(In19), LowerDist_n5/19(In19), LowerDist_n4/19(In19), LowerDist_n3/19(In19), LowerDist_n2/19(In19), LowerDist_n1/19(In19), Gateway Out24/1
  dist_k24/1 -> LowerDist_n44/24(In24), LowerDist_n47/24(In24), LowerDist_n49/24(In24), LowerDist_n48/24(In24), LowerDist_n46/24(In24), LowerDist_n45/24(In24), LowerDist_n43/24(In24), LowerDist_n42/24(In24), LowerDist_n41/24(In24), LowerDist_n31/24(In24), LowerDist_n34/24(In24), LowerDist_n37/24(In24), LowerDist_n40/24(In24), LowerDist_n39/24(In24), LowerDist_n38/24(In24), LowerDist_n36/24(In24), LowerDist_n35/24(In24), LowerDist_n33/24(In24), LowerDist_n32/24(In24), LowerDist_n27/24(In24), LowerDist_n30/24(In24), LowerDist_n29/24(In24), LowerDist_n28/24(In24), LowerDist_n26/24(In24), LowerDist_n25/24(In24), LowerDist_n24/1(In1), LowerDist_n23/24(In24), LowerDist_n22/24(In24), LowerDist_n21/24(In24), LowerDist_n17/24(In24), LowerDist_n20/24(In24), LowerDist_n19/24(In24), LowerDist_n18/24(In24), LowerDist_n16/24(In24), LowerDist_n15/24(In24), LowerDist_n14/24(In24), LowerDist_n13/24(In24), LowerDist_n12/24(In24), LowerDist_n11/24(In24), LowerDist_n7/24(In24), LowerDist_n10/24(In24), LowerDist_n9/24(In24), LowerDist_n8/24(In24), LowerDist_n6/24(In24), LowerDist_n5/24(In24), LowerDist_n4/24(In24), LowerDist_n3/24(In24), LowerDist_n2/24(In24), LowerDist_n1/24(In24), Gateway Out20/1
  dist_k2/1 -> LowerDist_n2/1(In1), LowerDist_n10/2(In2), LowerDist_n9/2(In2), LowerDist_n8/2(In2), LowerDist_n7/2(In2), LowerDist_n6/2(In2), LowerDist_n5/2(In2), LowerDist_n4/2(In2), LowerDist_n3/2(In2), LowerDist_n1/2(In2), LowerDist_n42/2(In2), LowerDist_n49/2(In2), LowerDist_n48/2(In2), LowerDist_n47/2(In2), LowerDist_n46/2(In2), LowerDist_n45/2(In2), LowerDist_n44/2(In2), LowerDist_n43/2(In2), LowerDist_n41/2(In2), LowerDist_n31/2(In2), LowerDist_n32/2(In2), LowerDist_n40/2(In2), LowerDist_n39/2(In2), LowerDist_n38/2(In2), LowerDist_n37/2(In2), LowerDist_n36/2(In2), LowerDist_n35/2(In2), LowerDist_n34/2(In2), LowerDist_n33/2(In2), LowerDist_n22/2(In2), LowerDist_n30/2(In2), LowerDist_n29/2(In2), LowerDist_n28/2(In2), LowerDist_n27/2(In2), LowerDist_n26/2(In2), LowerDist_n25/2(In2), LowerDist_n24/2(In2), LowerDist_n23/2(In2), LowerDist_n21/2(In2), LowerDist_n12/2(In2), LowerDist_n20/2(In2), LowerDist_n19/2(In2), LowerDist_n18/2(In2), LowerDist_n17/2(In2), LowerDist_n16/2(In2), LowerDist_n15/2(In2), LowerDist_n14/2(In2), LowerDist_n13/2(In2), LowerDist_n11/2(In2), Gateway Out1/1
  dist_k20/1 -> LowerDist_n10/20(In20), LowerDist_n9/20(In20), LowerDist_n8/20(In20), LowerDist_n7/20(In20), LowerDist_n6/20(In20), LowerDist_n5/20(In20), LowerDist_n4/20(In20), LowerDist_n3/20(In20), LowerDist_n2/20(In20), LowerDist_n1/20(In20), LowerDist_n20/1(In1), LowerDist_n19/20(In20), LowerDist_n18/20(In20), LowerDist_n17/20(In20), LowerDist_n16/20(In20), LowerDist_n15/20(In20), LowerDist_n14/20(In20), LowerDist_n13/20(In20), LowerDist_n12/20(In20), LowerDist_n11/20(In20), LowerDist_n30/20(In20), LowerDist_n29/20(In20), LowerDist_n28/20(In20), LowerDist_n27/20(In20), LowerDist_n26/20(In20), LowerDist_n25/20(In20), LowerDist_n24/20(In20), LowerDist_n23/20(In20), LowerDist_n22/20(In20), LowerDist_n21/20(In20), LowerDist_n49/20(In20), LowerDist_n48/20(In20), LowerDist_n47/20(In20), LowerDist_n46/20(In20), LowerDist_n45/20(In20), LowerDist_n44/20(In20), LowerDist_n43/20(In20), LowerDist_n42/20(In20), LowerDist_n41/20(In20), LowerDist_n31/20(In20), LowerDist_n40/20(In20), LowerDist_n39/20(In20), LowerDist_n38/20(In20), LowerDist_n37/20(In20), LowerDist_n36/20(In20), LowerDist_n35/20(In20), LowerDist_n34/20(In20), LowerDist_n33/20(In20), LowerDist_n32/20(In20), Gateway Out16/1
  dist_k26/1 -> LowerDist_n20/26(In26), LowerDist_n19/26(In26), LowerDist_n18/26(In26), LowerDist_n17/26(In26), LowerDist_n16/26(In26), LowerDist_n15/26(In26), LowerDist_n14/26(In26), LowerDist_n13/26(In26), LowerDist_n12/26(In26), LowerDist_n11/26(In26), LowerDist_n46/26(In26), LowerDist_n49/26(In26), LowerDist_n48/26(In26), LowerDist_n47/26(In26), LowerDist_n45/26(In26), LowerDist_n44/26(In26), LowerDist_n43/26(In26), LowerDist_n42/26(In26), LowerDist_n41/26(In26), LowerDist_n31/26(In26), LowerDist_n36/26(In26), LowerDist_n40/26(In26), LowerDist_n39/26(In26), LowerDist_n38/26(In26), LowerDist_n37/26(In26), LowerDist_n35/26(In26), LowerDist_n34/26(In26), LowerDist_n33/26(In26), LowerDist_n32/26(In26), LowerDist_n30/26(In26), LowerDist_n29/26(In26), LowerDist_n28/26(In26), LowerDist_n27/26(In26), LowerDist_n26/1(In1), LowerDist_n25/26(In26), LowerDist_n24/26(In26), LowerDist_n23/26(In26), LowerDist_n22/26(In26), LowerDist_n21/26(In26), LowerDist_n10/26(In26), LowerDist_n9/26(In26), LowerDist_n8/26(In26), LowerDist_n7/26(In26), LowerDist_n6/26(In26), LowerDist_n5/26(In26), LowerDist_n4/26(In26), LowerDist_n3/26(In26), LowerDist_n2/26(In26), LowerDist_n1/26(In26), Gateway Out25/1
  dist_k27/1 -> Gateway Out26/1, LowerDist_n20/27(In27), LowerDist_n19/27(In27), LowerDist_n18/27(In27), LowerDist_n17/27(In27), LowerDist_n16/27(In27), LowerDist_n15/27(In27), LowerDist_n14/27(In27), LowerDist_n13/27(In27), LowerDist_n12/27(In27), LowerDist_n11/27(In27), LowerDist_n47/27(In27), LowerDist_n49/27(In27), LowerDist_n48/27(In27), LowerDist_n46/27(In27), LowerDist_n45/27(In27), LowerDist_n44/27(In27), LowerDist_n43/27(In27), LowerDist_n42/27(In27), LowerDist_n41/27(In27), LowerDist_n31/27(In27), LowerDist_n37/27(In27), LowerDist_n40/27(In27), LowerDist_n39/27(In27), LowerDist_n38/27(In27), LowerDist_n36/27(In27), LowerDist_n35/27(In27), LowerDist_n34/27(In27), LowerDist_n33/27(In27), LowerDist_n32/27(In27), LowerDist_n30/27(In27), LowerDist_n29/27(In27), LowerDist_n28/27(In27), LowerDist_n27/1(In1), LowerDist_n26/27(In27), LowerDist_n25/27(In27), LowerDist_n24/27(In27), LowerDist_n23/27(In27), LowerDist_n22/27(In27), LowerDist_n21/27(In27), LowerDist_n10/27(In27), LowerDist_n9/27(In27), LowerDist_n8/27(In27), LowerDist_n7/27(In27), LowerDist_n6/27(In27), LowerDist_n5/27(In27), LowerDist_n4/27(In27), LowerDist_n3/27(In27), LowerDist_n2/27(In27), LowerDist_n1/27(In27)
  dist_k28/1 -> LowerDist_n1/28(In28), LowerDist_n2/28(In28), LowerDist_n3/28(In28), LowerDist_n4/28(In28), LowerDist_n5/28(In28), LowerDist_n6/28(In28), LowerDist_n7/28(In28), LowerDist_n8/28(In28), LowerDist_n10/28(In28), LowerDist_n9/28(In28), Gateway Out41/1, LowerDist_n11/28(In28), LowerDist_n13/28(In28), LowerDist_n14/28(In28), LowerDist_n15/28(In28), LowerDist_n16/28(In28), LowerDist_n20/28(In28), LowerDist_n19/28(In28), LowerDist_n18/28(In28), LowerDist_n17/28(In28), LowerDist_n12/28(In28), LowerDist_n41/28(In28), LowerDist_n42/28(In28), LowerDist_n43/28(In28), LowerDist_n44/28(In28), LowerDist_n46/28(In28), LowerDist_n47/28(In28), LowerDist_n48/28(In28), LowerDist_n49/28(In28), LowerDist_n45/28(In28), LowerDist_n31/28(In28), LowerDist_n32/28(In28), LowerDist_n33/28(In28), LowerDist_n34/28(In28), LowerDist_n36/28(In28), LowerDist_n37/28(In28), LowerDist_n38/28(In28), LowerDist_n40/28(In28), LowerDist_n39/28(In28), LowerDist_n35/28(In28), LowerDist_n21/28(In28), LowerDist_n22/28(In28), LowerDist_n23/28(In28), LowerDist_n24/28(In28), LowerDist_n26/28(In28), LowerDist_n27/28(In28), LowerDist_n30/28(In28), LowerDist_n29/28(In28), LowerDist_n28/1(In1), LowerDist_n25/28(In28)
  dist_k31/1 -> Gateway Out49/1, LowerDist_n41/31(In31), LowerDist_n49/31(In31), LowerDist_n48/31(In31), LowerDist_n47/31(In31), LowerDist_n46/31(In31), LowerDist_n45/31(In31), LowerDist_n44/31(In31), LowerDist_n43/31(In31), LowerDist_n42/31(In31), LowerDist_n31/1(In1), LowerDist_n40/31(In31), LowerDist_n39/31(In31), LowerDist_n38/31(In31), LowerDist_n37/31(In31), LowerDist_n36/31(In31), LowerDist_n35/31(In31), LowerDist_n34/31(In31), LowerDist_n33/31(In31), LowerDist_n32/31(In31), LowerDist_n30/31(In31), LowerDist_n29/31(In31), LowerDist_n28/31(In31), LowerDist_n27/31(In31), LowerDist_n26/31(In31), LowerDist_n25/31(In31), LowerDist_n24/31(In31), LowerDist_n23/31(In31), LowerDist_n22/31(In31), LowerDist_n21/31(In31), LowerDist_n20/31(In31), LowerDist_n19/31(In31), LowerDist_n18/31(In31), LowerDist_n17/31(In31), LowerDist_n16/31(In31), LowerDist_n15/31(In31), LowerDist_n14/31(In31), LowerDist_n13/31(In31), LowerDist_n12/31(In31), LowerDist_n11/31(In31), LowerDist_n10/31(In31), LowerDist_n9/31(In31), LowerDist_n8/31(In31), LowerDist_n7/31(In31), LowerDist_n6/31(In31), LowerDist_n5/31(In31), LowerDist_n4/31(In31), LowerDist_n3/31(In31), LowerDist_n2/31(In31), LowerDist_n1/31(In31)
  dist_k32/1 -> LowerDist_n10/32(In32), LowerDist_n9/32(In32), LowerDist_n8/32(In32), LowerDist_n7/32(In32), LowerDist_n6/32(In32), LowerDist_n5/32(In32), LowerDist_n4/32(In32), LowerDist_n3/32(In32), LowerDist_n2/32(In32), LowerDist_n1/32(In32), LowerDist_n42/32(In32), LowerDist_n49/32(In32), LowerDist_n48/32(In32), LowerDist_n47/32(In32), LowerDist_n46/32(In32), LowerDist_n45/32(In32), LowerDist_n44/32(In32), LowerDist_n43/32(In32), LowerDist_n41/32(In32), LowerDist_n31/32(In32), LowerDist_n40/32(In32), LowerDist_n39/32(In32), LowerDist_n38/32(In32), LowerDist_n37/32(In32), LowerDist_n36/32(In32), LowerDist_n35/32(In32), LowerDist_n34/32(In32), LowerDist_n33/32(In32), LowerDist_n32/1(In1), LowerDist_n30/32(In32), LowerDist_n29/32(In32), LowerDist_n28/32(In32), LowerDist_n27/32(In32), LowerDist_n26/32(In32), LowerDist_n25/32(In32), LowerDist_n24/32(In32), LowerDist_n23/32(In32), LowerDist_n22/32(In32), LowerDist_n21/32(In32), LowerDist_n20/32(In32), LowerDist_n19/32(In32), LowerDist_n18/32(In32), LowerDist_n17/32(In32), LowerDist_n16/32(In32), LowerDist_n15/32(In32), LowerDist_n14/32(In32), LowerDist_n13/32(In32), LowerDist_n12/32(In32), LowerDist_n11/32(In32), Gateway Out50/1
  dist_k33/1 -> LowerDist_n10/33(In33), LowerDist_n9/33(In33), LowerDist_n8/33(In33), LowerDist_n7/33(In33), LowerDist_n6/33(In33), LowerDist_n5/33(In33), LowerDist_n4/33(In33), LowerDist_n3/33(In33), LowerDist_n2/33(In33), LowerDist_n1/33(In33), LowerDist_n43/33(In33), LowerDist_n49/33(In33), LowerDist_n48/33(In33), LowerDist_n47/33(In33), LowerDist_n46/33(In33), LowerDist_n45/33(In33), LowerDist_n44/33(In33), LowerDist_n42/33(In33), LowerDist_n41/33(In33), LowerDist_n31/33(In33), LowerDist_n33/1(In1), LowerDist_n40/33(In33), LowerDist_n39/33(In33), LowerDist_n38/33(In33), LowerDist_n37/33(In33), LowerDist_n36/33(In33), LowerDist_n35/33(In33), LowerDist_n34/33(In33), LowerDist_n32/33(In33), LowerDist_n30/33(In33), LowerDist_n29/33(In33), LowerDist_n28/33(In33), LowerDist_n27/33(In33), LowerDist_n26/33(In33), LowerDist_n25/33(In33), LowerDist_n24/33(In33), LowerDist_n23/33(In33), LowerDist_n22/33(In33), LowerDist_n21/33(In33), LowerDist_n20/33(In33), LowerDist_n19/33(In33), LowerDist_n18/33(In33), LowerDist_n17/33(In33), LowerDist_n16/33(In33), LowerDist_n15/33(In33), LowerDist_n14/33(In33), LowerDist_n13/33(In33), LowerDist_n12/33(In33), LowerDist_n11/33(In33), Gateway Out51/1
  dist_k34/1 -> LowerDist_n44/34(In34), LowerDist_n49/34(In34), LowerDist_n48/34(In34), LowerDist_n47/34(In34), LowerDist_n46/34(In34), LowerDist_n45/34(In34), LowerDist_n43/34(In34), LowerDist_n42/34(In34), LowerDist_n41/34(In34), LowerDist_n31/34(In34), LowerDist_n40/34(In34), LowerDist_n39/34(In34), LowerDist_n38/34(In34), LowerDist_n37/34(In34), LowerDist_n36/34(In34), LowerDist_n35/34(In34), LowerDist_n34/1(In1), LowerDist_n33/34(In34), LowerDist_n32/34(In34), LowerDist_n30/34(In34), LowerDist_n29/34(In34), LowerDist_n28/34(In34), LowerDist_n27/34(In34), LowerDist_n26/34(In34), LowerDist_n25/34(In34), LowerDist_n24/34(In34), LowerDist_n23/34(In34), LowerDist_n22/34(In34), LowerDist_n21/34(In34), LowerDist_n20/34(In34), LowerDist_n19/34(In34), LowerDist_n18/34(In34), LowerDist_n17/34(In34), LowerDist_n16/34(In34), LowerDist_n15/34(In34), LowerDist_n14/34(In34), LowerDist_n13/34(In34), LowerDist_n12/34(In34), LowerDist_n11/34(In34), LowerDist_n10/34(In34), LowerDist_n9/34(In34), LowerDist_n8/34(In34), LowerDist_n7/34(In34), LowerDist_n6/34(In34), LowerDist_n5/34(In34), LowerDist_n4/34(In34), LowerDist_n3/34(In34), LowerDist_n2/34(In34), LowerDist_n1/34(In34), Gateway Out52/1
  dist_k35/1 -> LowerDist_n45/35(In35), LowerDist_n49/35(In35), LowerDist_n48/35(In35), LowerDist_n47/35(In35), LowerDist_n46/35(In35), LowerDist_n44/35(In35), LowerDist_n43/35(In35), LowerDist_n42/35(In35), LowerDist_n41/35(In35), LowerDist_n31/35(In35), LowerDist_n40/35(In35), LowerDist_n39/35(In35), LowerDist_n38/35(In35), LowerDist_n37/35(In35), LowerDist_n36/35(In35), LowerDist_n35/1(In1), LowerDist_n34/35(In35), LowerDist_n33/35(In35), LowerDist_n32/35(In35), LowerDist_n30/35(In35), LowerDist_n29/35(In35), LowerDist_n28/35(In35), LowerDist_n27/35(In35), LowerDist_n26/35(In35), LowerDist_n25/35(In35), LowerDist_n24/35(In35), LowerDist_n23/35(In35), LowerDist_n22/35(In35), LowerDist_n21/35(In35), LowerDist_n20/35(In35), LowerDist_n19/35(In35), LowerDist_n18/35(In35), LowerDist_n17/35(In35), LowerDist_n16/35(In35), LowerDist_n15/35(In35), LowerDist_n14/35(In35), LowerDist_n13/35(In35), LowerDist_n12/35(In35), LowerDist_n11/35(In35), LowerDist_n10/35(In35), LowerDist_n9/35(In35), LowerDist_n8/35(In35), LowerDist_n7/35(In35), LowerDist_n6/35(In35), LowerDist_n5/35(In35), LowerDist_n4/35(In35), LowerDist_n3/35(In35), LowerDist_n2/35(In35), LowerDist_n1/35(In35), Gateway Out53/1
  dist_k36/1 -> LowerDist_n7/36(In36), LowerDist_n10/36(In36), LowerDist_n9/36(In36), LowerDist_n8/36(In36), LowerDist_n6/36(In36), LowerDist_n5/36(In36), LowerDist_n4/36(In36), LowerDist_n3/36(In36), LowerDist_n2/36(In36), LowerDist_n1/36(In36), LowerDist_n27/36(In36), LowerDist_n30/36(In36), LowerDist_n29/36(In36), LowerDist_n28/36(In36), LowerDist_n26/36(In36), LowerDist_n25/36(In36), LowerDist_n24/36(In36), LowerDist_n23/36(In36), LowerDist_n22/36(In36), LowerDist_n21/36(In36), LowerDist_n46/36(In36), LowerDist_n47/36(In36), LowerDist_n49/36(In36), LowerDist_n48/36(In36), LowerDist_n45/36(In36), LowerDist_n44/36(In36), LowerDist_n43/36(In36), LowerDist_n42/36(In36), LowerDist_n41/36(In36), LowerDist_n31/36(In36), LowerDist_n37/36(In36), LowerDist_n40/36(In36), LowerDist_n39/36(In36), LowerDist_n38/36(In36), LowerDist_n36/1(In1), LowerDist_n35/36(In36), LowerDist_n34/36(In36), LowerDist_n33/36(In36), LowerDist_n32/36(In36), LowerDist_n17/36(In36), LowerDist_n20/36(In36), LowerDist_n19/36(In36), LowerDist_n18/36(In36), LowerDist_n16/36(In36), LowerDist_n15/36(In36), LowerDist_n14/36(In36), LowerDist_n13/36(In36), LowerDist_n12/36(In36), LowerDist_n11/36(In36), Gateway Out31/1
  dist_k37/1 -> LowerDist_n47/37(In37), LowerDist_n49/37(In37), LowerDist_n48/37(In37), LowerDist_n46/37(In37), LowerDist_n45/37(In37), LowerDist_n44/37(In37), LowerDist_n43/37(In37), LowerDist_n42/37(In37), LowerDist_n41/37(In37), LowerDist_n31/37(In37), LowerDist_n40/37(In37), LowerDist_n39/37(In37), LowerDist_n38/37(In37), LowerDist_n37/1(In1), LowerDist_n36/37(In37), LowerDist_n35/37(In37), LowerDist_n34/37(In37), LowerDist_n33/37(In37), LowerDist_n32/37(In37), LowerDist_n30/37(In37), LowerDist_n29/37(In37), LowerDist_n28/37(In37), LowerDist_n27/37(In37), LowerDist_n26/37(In37), LowerDist_n25/37(In37), LowerDist_n24/37(In37), LowerDist_n23/37(In37), LowerDist_n22/37(In37), LowerDist_n21/37(In37), LowerDist_n20/37(In37), LowerDist_n19/37(In37), LowerDist_n18/37(In37), LowerDist_n17/37(In37), LowerDist_n16/37(In37), LowerDist_n15/37(In37), LowerDist_n14/37(In37), LowerDist_n13/37(In37), LowerDist_n12/37(In37), LowerDist_n11/37(In37), LowerDist_n10/37(In37), LowerDist_n9/37(In37), LowerDist_n8/37(In37), LowerDist_n7/37(In37), LowerDist_n6/37(In37), LowerDist_n5/37(In37), LowerDist_n4/37(In37), LowerDist_n3/37(In37), LowerDist_n2/37(In37), LowerDist_n1/37(In37), Gateway Out32/1
  dist_k38/1 -> Gateway Out33/1, LowerDist_n48/38(In38), LowerDist_n49/38(In38), LowerDist_n47/38(In38), LowerDist_n46/38(In38), LowerDist_n45/38(In38), LowerDist_n44/38(In38), LowerDist_n43/38(In38), LowerDist_n42/38(In38), LowerDist_n41/38(In38), LowerDist_n31/38(In38), LowerDist_n40/38(In38), LowerDist_n39/38(In38), LowerDist_n38/1(In1), LowerDist_n37/38(In38), LowerDist_n36/38(In38), LowerDist_n35/38(In38), LowerDist_n34/38(In38), LowerDist_n33/38(In38), LowerDist_n32/38(In38), LowerDist_n30/38(In38), LowerDist_n29/38(In38), LowerDist_n28/38(In38), LowerDist_n27/38(In38), LowerDist_n26/38(In38), LowerDist_n25/38(In38), LowerDist_n24/38(In38), LowerDist_n23/38(In38), LowerDist_n22/38(In38), LowerDist_n21/38(In38), LowerDist_n20/38(In38), LowerDist_n19/38(In38), LowerDist_n18/38(In38), LowerDist_n17/38(In38), LowerDist_n16/38(In38), LowerDist_n15/38(In38), LowerDist_n14/38(In38), LowerDist_n13/38(In38), LowerDist_n12/38(In38), LowerDist_n11/38(In38), LowerDist_n10/38(In38), LowerDist_n9/38(In38), LowerDist_n8/38(In38), LowerDist_n7/38(In38), LowerDist_n6/38(In38), LowerDist_n5/38(In38), LowerDist_n4/38(In38), LowerDist_n3/38(In38), LowerDist_n2/38(In38), LowerDist_n1/38(In38)
  dist_k41/1 -> LowerDist_n10/41(In41), LowerDist_n9/41(In41), LowerDist_n8/41(In41), LowerDist_n7/41(In41), LowerDist_n6/41(In41), LowerDist_n5/41(In41), LowerDist_n4/41(In41), LowerDist_n3/41(In41), LowerDist_n2/41(In41), LowerDist_n1/41(In41), Gateway Out36/1, LowerDist_n30/41(In41), LowerDist_n29/41(In41), LowerDist_n28/41(In41), LowerDist_n27/41(In41), LowerDist_n26/41(In41), LowerDist_n25/41(In41), LowerDist_n24/41(In41), LowerDist_n23/41(In41), LowerDist_n22/41(In41), LowerDist_n21/41(In41), LowerDist_n41/1(In1), LowerDist_n49/41(In41), LowerDist_n48/41(In41), LowerDist_n47/41(In41), LowerDist_n46/41(In41), LowerDist_n45/41(In41), LowerDist_n44/41(In41), LowerDist_n43/41(In41), LowerDist_n42/41(In41), LowerDist_n31/41(In41), LowerDist_n40/41(In41), LowerDist_n39/41(In41), LowerDist_n38/41(In41), LowerDist_n37/41(In41), LowerDist_n36/41(In41), LowerDist_n35/41(In41), LowerDist_n34/41(In41), LowerDist_n33/41(In41), LowerDist_n32/41(In41), LowerDist_n20/41(In41), LowerDist_n19/41(In41), LowerDist_n18/41(In41), LowerDist_n17/41(In41), LowerDist_n16/41(In41), LowerDist_n15/41(In41), LowerDist_n14/41(In41), LowerDist_n13/41(In41), LowerDist_n12/41(In41), LowerDist_n11/41(In41)
  dist_k42/1 -> LowerDist_n28/42(In42), LowerDist_n30/42(In42), LowerDist_n29/42(In42), LowerDist_n27/42(In42), LowerDist_n26/42(In42), LowerDist_n25/42(In42), LowerDist_n24/42(In42), LowerDist_n23/42(In42), LowerDist_n22/42(In42), LowerDist_n21/42(In42), LowerDist_n42/1(In1), LowerDist_n48/42(In42), LowerDist_n49/42(In42), LowerDist_n47/42(In42), LowerDist_n46/42(In42), LowerDist_n45/42(In42), LowerDist_n44/42(In42), LowerDist_n43/42(In42), LowerDist_n41/42(In42), LowerDist_n31/42(In42), LowerDist_n38/42(In42), LowerDist_n40/42(In42), LowerDist_n39/42(In42), LowerDist_n37/42(In42), LowerDist_n36/42(In42), LowerDist_n35/42(In42), LowerDist_n34/42(In42), LowerDist_n33/42(In42), LowerDist_n32/42(In42), LowerDist_n18/42(In42), LowerDist_n20/42(In42), LowerDist_n19/42(In42), LowerDist_n17/42(In42), LowerDist_n16/42(In42), LowerDist_n15/42(In42), LowerDist_n14/42(In42), LowerDist_n13/42(In42), LowerDist_n12/42(In42), LowerDist_n11/42(In42), LowerDist_n8/42(In42), LowerDist_n10/42(In42), LowerDist_n9/42(In42), LowerDist_n7/42(In42), LowerDist_n6/42(In42), LowerDist_n5/42(In42), LowerDist_n4/42(In42), LowerDist_n3/42(In42), LowerDist_n2/42(In42), LowerDist_n1/42(In42), Gateway Out44/1
  dist_k43/1 -> LowerDist_n7/43(In43), LowerDist_n10/43(In43), LowerDist_n9/43(In43), LowerDist_n8/43(In43), LowerDist_n6/43(In43), LowerDist_n5/43(In43), LowerDist_n4/43(In43), LowerDist_n3/43(In43), LowerDist_n2/43(In43), LowerDist_n1/43(In43), LowerDist_n27/43(In43), LowerDist_n30/43(In43), LowerDist_n29/43(In43), LowerDist_n28/43(In43), LowerDist_n26/43(In43), LowerDist_n25/43(In43), LowerDist_n24/43(In43), LowerDist_n23/43(In43), LowerDist_n22/43(In43), LowerDist_n21/43(In43), LowerDist_n47/43(In43), LowerDist_n49/43(In43), LowerDist_n48/43(In43), LowerDist_n46/43(In43), LowerDist_n45/43(In43), LowerDist_n44/43(In43), LowerDist_n43/1(In1), LowerDist_n42/43(In43), LowerDist_n41/43(In43), LowerDist_n31/43(In43), LowerDist_n37/43(In43), LowerDist_n40/43(In43), LowerDist_n39/43(In43), LowerDist_n38/43(In43), LowerDist_n36/43(In43), LowerDist_n35/43(In43), LowerDist_n34/43(In43), LowerDist_n33/43(In43), LowerDist_n32/43(In43), LowerDist_n17/43(In43), LowerDist_n20/43(In43), LowerDist_n19/43(In43), LowerDist_n18/43(In43), LowerDist_n16/43(In43), LowerDist_n15/43(In43), LowerDist_n14/43(In43), LowerDist_n13/43(In43), LowerDist_n12/43(In43), LowerDist_n11/43(In43), Gateway Out45/1
  dist_k44/1 -> LowerDist_n44/1(In1), LowerDist_n49/44(In44), LowerDist_n48/44(In44), LowerDist_n47/44(In44), LowerDist_n46/44(In44), LowerDist_n45/44(In44), LowerDist_n43/44(In44), LowerDist_n42/44(In44), LowerDist_n41/44(In44), LowerDist_n31/44(In44), LowerDist_n40/44(In44), LowerDist_n39/44(In44), LowerDist_n38/44(In44), LowerDist_n37/44(In44), LowerDist_n36/44(In44), LowerDist_n35/44(In44), LowerDist_n34/44(In44), LowerDist_n33/44(In44), LowerDist_n32/44(In44), LowerDist_n30/44(In44), LowerDist_n29/44(In44), LowerDist_n28/44(In44), LowerDist_n27/44(In44), LowerDist_n26/44(In44), LowerDist_n25/44(In44), LowerDist_n24/44(In44), LowerDist_n23/44(In44), LowerDist_n22/44(In44), LowerDist_n21/44(In44), LowerDist_n20/44(In44), LowerDist_n19/44(In44), LowerDist_n18/44(In44), LowerDist_n17/44(In44), LowerDist_n16/44(In44), LowerDist_n15/44(In44), LowerDist_n14/44(In44), LowerDist_n13/44(In44), LowerDist_n12/44(In44), LowerDist_n11/44(In44), LowerDist_n10/44(In44), LowerDist_n9/44(In44), LowerDist_n8/44(In44), LowerDist_n7/44(In44), LowerDist_n6/44(In44), LowerDist_n5/44(In44), LowerDist_n4/44(In44), LowerDist_n3/44(In44), LowerDist_n2/44(In44), LowerDist_n1/44(In44), Gateway Out46/1
  dist_k45/1 -> LowerDist_n10/45(In45), LowerDist_n9/45(In45), LowerDist_n8/45(In45), LowerDist_n7/45(In45), LowerDist_n6/45(In45), LowerDist_n5/45(In45), LowerDist_n4/45(In45), LowerDist_n3/45(In45), LowerDist_n2/45(In45), LowerDist_n1/45(In45), LowerDist_n49/45(In45), LowerDist_n48/45(In45), LowerDist_n47/45(In45), LowerDist_n46/45(In45), LowerDist_n45/1(In1), LowerDist_n44/45(In45), LowerDist_n43/45(In45), LowerDist_n42/45(In45), LowerDist_n41/45(In45), LowerDist_n31/45(In45), LowerDist_n40/45(In45), LowerDist_n39/45(In45), LowerDist_n38/45(In45), LowerDist_n37/45(In45), LowerDist_n36/45(In45), LowerDist_n35/45(In45), LowerDist_n34/45(In45), LowerDist_n33/45(In45), LowerDist_n32/45(In45), LowerDist_n30/45(In45), LowerDist_n29/45(In45), LowerDist_n28/45(In45), LowerDist_n27/45(In45), LowerDist_n26/45(In45), LowerDist_n25/45(In45), LowerDist_n24/45(In45), LowerDist_n23/45(In45), LowerDist_n22/45(In45), LowerDist_n21/45(In45), LowerDist_n20/45(In45), LowerDist_n19/45(In45), LowerDist_n18/45(In45), LowerDist_n17/45(In45), LowerDist_n16/45(In45), LowerDist_n15/45(In45), LowerDist_n14/45(In45), LowerDist_n13/45(In45), LowerDist_n12/45(In45), LowerDist_n11/45(In45), Gateway Out37/1
  dist_k46/1 -> LowerDist_n10/46(In46), LowerDist_n9/46(In46), LowerDist_n8/46(In46), LowerDist_n7/46(In46), LowerDist_n6/46(In46), LowerDist_n5/46(In46), LowerDist_n4/46(In46), LowerDist_n3/46(In46), LowerDist_n2/46(In46), LowerDist_n1/46(In46), LowerDist_n49/46(In46), LowerDist_n48/46(In46), LowerDist_n47/46(In46), LowerDist_n46/1(In1), LowerDist_n45/46(In46), LowerDist_n44/46(In46), LowerDist_n43/46(In46), LowerDist_n42/46(In46), LowerDist_n41/46(In46), LowerDist_n31/46(In46), LowerDist_n40/46(In46), LowerDist_n39/46(In46), LowerDist_n38/46(In46), LowerDist_n37/46(In46), LowerDist_n36/46(In46), LowerDist_n35/46(In46), LowerDist_n34/46(In46), LowerDist_n33/46(In46), LowerDist_n32/46(In46), LowerDist_n30/46(In46), LowerDist_n29/46(In46), LowerDist_n28/46(In46), LowerDist_n27/46(In46), LowerDist_n26/46(In46), LowerDist_n25/46(In46), LowerDist_n24/46(In46), LowerDist_n23/46(In46), LowerDist_n22/46(In46), LowerDist_n21/46(In46), LowerDist_n20/46(In46), LowerDist_n19/46(In46), LowerDist_n18/46(In46), LowerDist_n17/46(In46), LowerDist_n16/46(In46), LowerDist_n15/46(In46), LowerDist_n14/46(In46), LowerDist_n13/46(In46), LowerDist_n12/46(In46), LowerDist_n11/46(In46), Gateway Out38/1
  dist_k48/1 -> LowerDist_n20/48(In48), LowerDist_n19/48(In48), LowerDist_n18/48(In48), LowerDist_n17/48(In48), LowerDist_n16/48(In48), LowerDist_n15/48(In48), LowerDist_n14/48(In48), LowerDist_n13/48(In48), LowerDist_n12/48(In48), LowerDist_n11/48(In48), LowerDist_n30/48(In48), LowerDist_n29/48(In48), LowerDist_n28/48(In48), LowerDist_n27/48(In48), LowerDist_n26/48(In48), LowerDist_n25/48(In48), LowerDist_n24/48(In48), LowerDist_n23/48(In48), LowerDist_n22/48(In48), LowerDist_n21/48(In48), LowerDist_n49/48(In48), LowerDist_n48/1(In1), LowerDist_n47/48(In48), LowerDist_n46/48(In48), LowerDist_n45/48(In48), LowerDist_n44/48(In48), LowerDist_n43/48(In48), LowerDist_n42/48(In48), LowerDist_n41/48(In48), LowerDist_n31/48(In48), LowerDist_n40/48(In48), LowerDist_n39/48(In48), LowerDist_n38/48(In48), LowerDist_n37/48(In48), LowerDist_n36/48(In48), LowerDist_n35/48(In48), LowerDist_n34/48(In48), LowerDist_n33/48(In48), LowerDist_n32/48(In48), LowerDist_n10/48(In48), LowerDist_n9/48(In48), LowerDist_n8/48(In48), LowerDist_n7/48(In48), LowerDist_n6/48(In48), LowerDist_n5/48(In48), LowerDist_n4/48(In48), LowerDist_n3/48(In48), LowerDist_n2/48(In48), LowerDist_n1/48(In48), Gateway Out40/1
  dist_k10/1 -> LowerDist_n12/10(In10), LowerDist_n20/10(In10), LowerDist_n19/10(In10), LowerDist_n18/10(In10), LowerDist_n17/10(In10), LowerDist_n16/10(In10), LowerDist_n15/10(In10), LowerDist_n14/10(In10), LowerDist_n13/10(In10), LowerDist_n11/10(In10), LowerDist_n21/10(In10), LowerDist_n22/10(In10), LowerDist_n30/10(In10), LowerDist_n29/10(In10), LowerDist_n28/10(In10), LowerDist_n27/10(In10), LowerDist_n26/10(In10), LowerDist_n25/10(In10), LowerDist_n24/10(In10), LowerDist_n23/10(In10), LowerDist_n41/10(In10), LowerDist_n42/10(In10), LowerDist_n49/10(In10), LowerDist_n48/10(In10), LowerDist_n47/10(In10), LowerDist_n46/10(In10), LowerDist_n45/10(In10), LowerDist_n44/10(In10), LowerDist_n43/10(In10), LowerDist_n31/10(In10), LowerDist_n32/10(In10), LowerDist_n40/10(In10), LowerDist_n39/10(In10), LowerDist_n38/10(In10), LowerDist_n37/10(In10), LowerDist_n36/10(In10), LowerDist_n35/10(In10), LowerDist_n34/10(In10), LowerDist_n33/10(In10), LowerDist_n10/1(In1), LowerDist_n9/10(In10), LowerDist_n8/10(In10), LowerDist_n7/10(In10), LowerDist_n6/10(In10), LowerDist_n5/10(In10), LowerDist_n4/10(In10), LowerDist_n3/10(In10), LowerDist_n2/10(In10), LowerDist_n1/10(In10), Gateway Out9/1
  dist_k6/1 -> LowerDist_n6/1(In1), LowerDist_n10/6(In6), LowerDist_n9/6(In6), LowerDist_n8/6(In6), LowerDist_n7/6(In6), LowerDist_n5/6(In6), LowerDist_n4/6(In6), LowerDist_n3/6(In6), LowerDist_n2/6(In6), LowerDist_n1/6(In6), LowerDist_n12/6(In6), LowerDist_n16/6(In6), LowerDist_n20/6(In6), LowerDist_n19/6(In6), LowerDist_n18/6(In6), LowerDist_n17/6(In6), LowerDist_n15/6(In6), LowerDist_n14/6(In6), LowerDist_n13/6(In6), LowerDist_n11/6(In6), LowerDist_n42/6(In6), LowerDist_n46/6(In6), LowerDist_n49/6(In6), LowerDist_n48/6(In6), LowerDist_n47/6(In6), LowerDist_n45/6(In6), LowerDist_n44/6(In6), LowerDist_n43/6(In6), LowerDist_n41/6(In6), LowerDist_n31/6(In6), LowerDist_n32/6(In6), LowerDist_n36/6(In6), LowerDist_n40/6(In6), LowerDist_n39/6(In6), LowerDist_n38/6(In6), LowerDist_n37/6(In6), LowerDist_n35/6(In6), LowerDist_n34/6(In6), LowerDist_n33/6(In6), LowerDist_n22/6(In6), LowerDist_n26/6(In6), LowerDist_n30/6(In6), LowerDist_n29/6(In6), LowerDist_n28/6(In6), LowerDist_n27/6(In6), LowerDist_n25/6(In6), LowerDist_n24/6(In6), LowerDist_n23/6(In6), LowerDist_n21/6(In6), Gateway Out5/1
  dist_k12/1 -> LowerDist_n10/12(In12), LowerDist_n9/12(In12), LowerDist_n8/12(In12), LowerDist_n7/12(In12), LowerDist_n6/12(In12), LowerDist_n5/12(In12), LowerDist_n4/12(In12), LowerDist_n3/12(In12), LowerDist_n2/12(In12), LowerDist_n1/12(In12), LowerDist_n20/12(In12), LowerDist_n19/12(In12), LowerDist_n18/12(In12), LowerDist_n17/12(In12), LowerDist_n16/12(In12), LowerDist_n15/12(In12), LowerDist_n14/12(In12), LowerDist_n13/12(In12), LowerDist_n12/1(In1), LowerDist_n11/12(In12), LowerDist_n21/12(In12), LowerDist_n22/12(In12), LowerDist_n30/12(In12), LowerDist_n29/12(In12), LowerDist_n28/12(In12), LowerDist_n27/12(In12), LowerDist_n26/12(In12), LowerDist_n25/12(In12), LowerDist_n24/12(In12), LowerDist_n23/12(In12), LowerDist_n41/12(In12), LowerDist_n42/12(In12), LowerDist_n49/12(In12), LowerDist_n48/12(In12), LowerDist_n47/12(In12), LowerDist_n46/12(In12), LowerDist_n45/12(In12), LowerDist_n44/12(In12), LowerDist_n43/12(In12), LowerDist_n31/12(In12), LowerDist_n32/12(In12), LowerDist_n40/12(In12), LowerDist_n39/12(In12), LowerDist_n38/12(In12), LowerDist_n37/12(In12), LowerDist_n36/12(In12), LowerDist_n35/12(In12), LowerDist_n34/12(In12), LowerDist_n33/12(In12), Gateway Out11/1
  dist_k40/1 -> LowerDist_n49/40(In40), LowerDist_n48/40(In40), LowerDist_n47/40(In40), LowerDist_n46/40(In40), LowerDist_n45/40(In40), LowerDist_n44/40(In40), LowerDist_n43/40(In40), LowerDist_n42/40(In40), LowerDist_n41/40(In40), LowerDist_n31/40(In40), LowerDist_n40/1(In1), LowerDist_n39/40(In40), LowerDist_n38/40(In40), LowerDist_n37/40(In40), LowerDist_n36/40(In40), LowerDist_n35/40(In40), LowerDist_n34/40(In40), LowerDist_n33/40(In40), LowerDist_n32/40(In40), LowerDist_n30/40(In40), LowerDist_n29/40(In40), LowerDist_n28/40(In40), LowerDist_n27/40(In40), LowerDist_n26/40(In40), LowerDist_n25/40(In40), LowerDist_n24/40(In40), LowerDist_n23/40(In40), LowerDist_n22/40(In40), LowerDist_n21/40(In40), LowerDist_n20/40(In40), LowerDist_n19/40(In40), LowerDist_n18/40(In40), LowerDist_n17/40(In40), LowerDist_n16/40(In40), LowerDist_n15/40(In40), LowerDist_n14/40(In40), LowerDist_n13/40(In40), LowerDist_n12/40(In40), LowerDist_n11/40(In40), LowerDist_n10/40(In40), LowerDist_n9/40(In40), LowerDist_n8/40(In40), LowerDist_n7/40(In40), LowerDist_n6/40(In40), LowerDist_n5/40(In40), LowerDist_n4/40(In40), LowerDist_n3/40(In40), LowerDist_n2/40(In40), LowerDist_n1/40(In40), Gateway Out35/1
  dist_k8/1 -> LowerDist_n22/8(In8), LowerDist_n28/8(In8), LowerDist_n30/8(In8), LowerDist_n29/8(In8), LowerDist_n27/8(In8), LowerDist_n26/8(In8), LowerDist_n25/8(In8), LowerDist_n24/8(In8), LowerDist_n23/8(In8), LowerDist_n21/8(In8), LowerDist_n42/8(In8), LowerDist_n48/8(In8), LowerDist_n49/8(In8), LowerDist_n47/8(In8), LowerDist_n46/8(In8), LowerDist_n45/8(In8), LowerDist_n44/8(In8), LowerDist_n43/8(In8), LowerDist_n41/8(In8), LowerDist_n31/8(In8), LowerDist_n32/8(In8), LowerDist_n38/8(In8), LowerDist_n40/8(In8), LowerDist_n39/8(In8), LowerDist_n37/8(In8), LowerDist_n36/8(In8), LowerDist_n35/8(In8), LowerDist_n34/8(In8), LowerDist_n33/8(In8), LowerDist_n12/8(In8), LowerDist_n18/8(In8), LowerDist_n20/8(In8), LowerDist_n19/8(In8), LowerDist_n17/8(In8), LowerDist_n16/8(In8), LowerDist_n15/8(In8), LowerDist_n14/8(In8), LowerDist_n13/8(In8), LowerDist_n11/8(In8), LowerDist_n8/1(In1), LowerDist_n10/8(In8), LowerDist_n9/8(In8), LowerDist_n7/8(In8), LowerDist_n6/8(In8), LowerDist_n5/8(In8), LowerDist_n4/8(In8), LowerDist_n3/8(In8), LowerDist_n2/8(In8), LowerDist_n1/8(In8), Gateway Out7/1
  dist_k5/1 -> LowerDist_n5/1(In1), LowerDist_n10/5(In5), LowerDist_n9/5(In5), LowerDist_n8/5(In5), LowerDist_n7/5(In5), LowerDist_n6/5(In5), LowerDist_n4/5(In5), LowerDist_n3/5(In5), LowerDist_n2/5(In5), LowerDist_n1/5(In5), LowerDist_n12/5(In5), LowerDist_n15/5(In5), LowerDist_n20/5(In5), LowerDist_n19/5(In5), LowerDist_n18/5(In5), LowerDist_n17/5(In5), LowerDist_n16/5(In5), LowerDist_n14/5(In5), LowerDist_n13/5(In5), LowerDist_n11/5(In5), LowerDist_n42/5(In5), LowerDist_n45/5(In5), LowerDist_n49/5(In5), LowerDist_n48/5(In5), LowerDist_n47/5(In5), LowerDist_n46/5(In5), LowerDist_n44/5(In5), LowerDist_n43/5(In5), LowerDist_n41/5(In5), LowerDist_n31/5(In5), LowerDist_n32/5(In5), LowerDist_n35/5(In5), LowerDist_n40/5(In5), LowerDist_n39/5(In5), LowerDist_n38/5(In5), LowerDist_n37/5(In5), LowerDist_n36/5(In5), LowerDist_n34/5(In5), LowerDist_n33/5(In5), LowerDist_n22/5(In5), LowerDist_n25/5(In5), LowerDist_n30/5(In5), LowerDist_n29/5(In5), LowerDist_n28/5(In5), LowerDist_n27/5(In5), LowerDist_n26/5(In5), LowerDist_n24/5(In5), LowerDist_n23/5(In5), LowerDist_n21/5(In5), Gateway Out4/1
  dist_k16/1 -> LowerDist_n10/16(In16), LowerDist_n9/16(In16), LowerDist_n8/16(In16), LowerDist_n7/16(In16), LowerDist_n6/16(In16), LowerDist_n5/16(In16), LowerDist_n4/16(In16), LowerDist_n3/16(In16), LowerDist_n2/16(In16), LowerDist_n1/16(In16), LowerDist_n20/16(In16), LowerDist_n19/16(In16), LowerDist_n18/16(In16), LowerDist_n17/16(In16), LowerDist_n16/1(In1), LowerDist_n15/16(In16), LowerDist_n14/16(In16), LowerDist_n13/16(In16), LowerDist_n12/16(In16), LowerDist_n11/16(In16), LowerDist_n26/16(In16), LowerDist_n30/16(In16), LowerDist_n29/16(In16), LowerDist_n28/16(In16), LowerDist_n27/16(In16), LowerDist_n25/16(In16), LowerDist_n24/16(In16), LowerDist_n23/16(In16), LowerDist_n22/16(In16), LowerDist_n21/16(In16), LowerDist_n46/16(In16), LowerDist_n49/16(In16), LowerDist_n48/16(In16), LowerDist_n47/16(In16), LowerDist_n45/16(In16), LowerDist_n44/16(In16), LowerDist_n43/16(In16), LowerDist_n42/16(In16), LowerDist_n41/16(In16), LowerDist_n31/16(In16), LowerDist_n36/16(In16), LowerDist_n40/16(In16), LowerDist_n39/16(In16), LowerDist_n38/16(In16), LowerDist_n37/16(In16), LowerDist_n35/16(In16), LowerDist_n34/16(In16), LowerDist_n33/16(In16), LowerDist_n32/16(In16), Gateway Out15/1
  dist_k30/1 -> LowerDist_n1/30(In30), LowerDist_n2/30(In30), LowerDist_n3/30(In30), LowerDist_n4/30(In30), LowerDist_n5/30(In30), LowerDist_n6/30(In30), LowerDist_n7/30(In30), LowerDist_n8/30(In30), LowerDist_n10/30(In30), LowerDist_n9/30(In30), LowerDist_n41/30(In30), LowerDist_n42/30(In30), LowerDist_n43/30(In30), LowerDist_n44/30(In30), LowerDist_n45/30(In30), LowerDist_n46/30(In30), LowerDist_n47/30(In30), LowerDist_n48/30(In30), LowerDist_n49/30(In30), LowerDist_n31/30(In30), LowerDist_n32/30(In30), LowerDist_n33/30(In30), LowerDist_n34/30(In30), LowerDist_n35/30(In30), LowerDist_n36/30(In30), LowerDist_n37/30(In30), LowerDist_n38/30(In30), LowerDist_n40/30(In30), LowerDist_n39/30(In30), LowerDist_n21/30(In30), LowerDist_n22/30(In30), LowerDist_n23/30(In30), LowerDist_n24/30(In30), LowerDist_n25/30(In30), LowerDist_n26/30(In30), LowerDist_n27/30(In30), LowerDist_n28/30(In30), LowerDist_n30/1(In1), LowerDist_n29/30(In30), LowerDist_n11/30(In30), LowerDist_n12/30(In30), LowerDist_n13/30(In30), LowerDist_n14/30(In30), LowerDist_n15/30(In30), LowerDist_n16/30(In30), LowerDist_n17/30(In30), LowerDist_n18/30(In30), LowerDist_n19/30(In30), LowerDist_n20/30(In30), Gateway Out48/1
  dist_k29/1 -> LowerDist_n1/29(In29), LowerDist_n2/29(In29), LowerDist_n3/29(In29), LowerDist_n4/29(In29), LowerDist_n5/29(In29), LowerDist_n6/29(In29), LowerDist_n7/29(In29), LowerDist_n8/29(In29), LowerDist_n10/29(In29), LowerDist_n9/29(In29), Gateway Out47/1, LowerDist_n11/29(In29), LowerDist_n13/29(In29), LowerDist_n14/29(In29), LowerDist_n16/29(In29), LowerDist_n17/29(In29), LowerDist_n18/29(In29), LowerDist_n20/29(In29), LowerDist_n19/29(In29), LowerDist_n15/29(In29), LowerDist_n12/29(In29), LowerDist_n41/29(In29), LowerDist_n42/29(In29), LowerDist_n43/29(In29), LowerDist_n44/29(In29), LowerDist_n45/29(In29), LowerDist_n46/29(In29), LowerDist_n47/29(In29), LowerDist_n48/29(In29), LowerDist_n49/29(In29), LowerDist_n31/29(In29), LowerDist_n32/29(In29), LowerDist_n33/29(In29), LowerDist_n34/29(In29), LowerDist_n35/29(In29), LowerDist_n36/29(In29), LowerDist_n37/29(In29), LowerDist_n38/29(In29), LowerDist_n39/29(In29), LowerDist_n40/29(In29), LowerDist_n21/29(In29), LowerDist_n22/29(In29), LowerDist_n23/29(In29), LowerDist_n24/29(In29), LowerDist_n25/29(In29), LowerDist_n26/29(In29), LowerDist_n27/29(In29), LowerDist_n28/29(In29), LowerDist_n29/1(In1), LowerDist_n30/29(In29)
  dist_k21/1 -> LowerDist_n10/21(In21), LowerDist_n9/21(In21), LowerDist_n8/21(In21), LowerDist_n7/21(In21), LowerDist_n6/21(In21), LowerDist_n5/21(In21), LowerDist_n4/21(In21), LowerDist_n3/21(In21), LowerDist_n2/21(In21), LowerDist_n1/21(In21), LowerDist_n20/21(In21), LowerDist_n19/21(In21), LowerDist_n18/21(In21), LowerDist_n17/21(In21), LowerDist_n16/21(In21), LowerDist_n15/21(In21), LowerDist_n14/21(In21), LowerDist_n13/21(In21), LowerDist_n12/21(In21), LowerDist_n11/21(In21), LowerDist_n41/21(In21), LowerDist_n49/21(In21), LowerDist_n48/21(In21), LowerDist_n47/21(In21), LowerDist_n46/21(In21), LowerDist_n45/21(In21), LowerDist_n44/21(In21), LowerDist_n43/21(In21), LowerDist_n42/21(In21), LowerDist_n31/21(In21), LowerDist_n40/21(In21), LowerDist_n39/21(In21), LowerDist_n38/21(In21), LowerDist_n37/21(In21), LowerDist_n36/21(In21), LowerDist_n35/21(In21), LowerDist_n34/21(In21), LowerDist_n33/21(In21), LowerDist_n32/21(In21), LowerDist_n30/21(In21), LowerDist_n29/21(In21), LowerDist_n28/21(In21), LowerDist_n27/21(In21), LowerDist_n26/21(In21), LowerDist_n25/21(In21), LowerDist_n24/21(In21), LowerDist_n23/21(In21), LowerDist_n22/21(In21), LowerDist_n21/1(In1), Gateway Out17/1
  dist_k22/1 -> LowerDist_n12/22(In22), LowerDist_n20/22(In22), LowerDist_n19/22(In22), LowerDist_n18/22(In22), LowerDist_n17/22(In22), LowerDist_n16/22(In22), LowerDist_n15/22(In22), LowerDist_n14/22(In22), LowerDist_n13/22(In22), LowerDist_n11/22(In22), LowerDist_n42/22(In22), LowerDist_n49/22(In22), LowerDist_n48/22(In22), LowerDist_n47/22(In22), LowerDist_n46/22(In22), LowerDist_n45/22(In22), LowerDist_n44/22(In22), LowerDist_n43/22(In22), LowerDist_n41/22(In22), LowerDist_n31/22(In22), LowerDist_n32/22(In22), LowerDist_n40/22(In22), LowerDist_n39/22(In22), LowerDist_n38/22(In22), LowerDist_n37/22(In22), LowerDist_n36/22(In22), LowerDist_n35/22(In22), LowerDist_n34/22(In22), LowerDist_n33/22(In22), LowerDist_n30/22(In22), LowerDist_n29/22(In22), LowerDist_n28/22(In22), LowerDist_n27/22(In22), LowerDist_n26/22(In22), LowerDist_n25/22(In22), LowerDist_n24/22(In22), LowerDist_n23/22(In22), LowerDist_n22/1(In1), LowerDist_n21/22(In22), LowerDist_n2/22(In22), LowerDist_n10/22(In22), LowerDist_n9/22(In22), LowerDist_n8/22(In22), LowerDist_n7/22(In22), LowerDist_n6/22(In22), LowerDist_n5/22(In22), LowerDist_n4/22(In22), LowerDist_n3/22(In22), LowerDist_n1/22(In22), Gateway Out18/1
  dist_k23/1 -> Gateway Out19/1, LowerDist_n43/23(In23), LowerDist_n49/23(In23), LowerDist_n48/23(In23), LowerDist_n47/23(In23), LowerDist_n46/23(In23), LowerDist_n45/23(In23), LowerDist_n44/23(In23), LowerDist_n42/23(In23), LowerDist_n41/23(In23), LowerDist_n31/23(In23), LowerDist_n33/23(In23), LowerDist_n40/23(In23), LowerDist_n39/23(In23), LowerDist_n38/23(In23), LowerDist_n37/23(In23), LowerDist_n36/23(In23), LowerDist_n35/23(In23), LowerDist_n34/23(In23), LowerDist_n32/23(In23), LowerDist_n30/23(In23), LowerDist_n29/23(In23), LowerDist_n28/23(In23), LowerDist_n27/23(In23), LowerDist_n26/23(In23), LowerDist_n25/23(In23), LowerDist_n24/23(In23), LowerDist_n23/1(In1), LowerDist_n22/23(In23), LowerDist_n21/23(In23), LowerDist_n20/23(In23), LowerDist_n19/23(In23), LowerDist_n18/23(In23), LowerDist_n17/23(In23), LowerDist_n16/23(In23), LowerDist_n15/23(In23), LowerDist_n14/23(In23), LowerDist_n13/23(In23), LowerDist_n12/23(In23), LowerDist_n11/23(In23), LowerDist_n10/23(In23), LowerDist_n9/23(In23), LowerDist_n8/23(In23), LowerDist_n7/23(In23), LowerDist_n6/23(In23), LowerDist_n5/23(In23), LowerDist_n4/23(In23), LowerDist_n3/23(In23), LowerDist_n2/23(In23), LowerDist_n1/23(In23)
  dist_k39/1 -> LowerDist_n30/39(In39), LowerDist_n29/39(In39), LowerDist_n28/39(In39), LowerDist_n27/39(In39), LowerDist_n26/39(In39), LowerDist_n25/39(In39), LowerDist_n24/39(In39), LowerDist_n23/39(In39), LowerDist_n22/39(In39), LowerDist_n21/39(In39), LowerDist_n49/39(In39), LowerDist_n48/39(In39), LowerDist_n47/39(In39), LowerDist_n46/39(In39), LowerDist_n45/39(In39), LowerDist_n44/39(In39), LowerDist_n43/39(In39), LowerDist_n42/39(In39), LowerDist_n41/39(In39), LowerDist_n31/39(In39), LowerDist_n40/39(In39), LowerDist_n39/1(In1), LowerDist_n38/39(In39), LowerDist_n37/39(In39), LowerDist_n36/39(In39), LowerDist_n35/39(In39), LowerDist_n34/39(In39), LowerDist_n33/39(In39), LowerDist_n32/39(In39), LowerDist_n20/39(In39), LowerDist_n19/39(In39), LowerDist_n18/39(In39), LowerDist_n17/39(In39), LowerDist_n16/39(In39), LowerDist_n15/39(In39), LowerDist_n14/39(In39), LowerDist_n13/39(In39), LowerDist_n12/39(In39), LowerDist_n11/39(In39), LowerDist_n10/39(In39), LowerDist_n9/39(In39), LowerDist_n8/39(In39), LowerDist_n7/39(In39), LowerDist_n6/39(In39), LowerDist_n5/39(In39), LowerDist_n4/39(In39), LowerDist_n3/39(In39), LowerDist_n2/39(In39), LowerDist_n1/39(In39), Gateway Out34/1
  dist_k47/1 -> LowerDist_n30/47(In47), LowerDist_n29/47(In47), LowerDist_n28/47(In47), LowerDist_n27/47(In47), LowerDist_n26/47(In47), LowerDist_n25/47(In47), LowerDist_n24/47(In47), LowerDist_n23/47(In47), LowerDist_n22/47(In47), LowerDist_n21/47(In47), LowerDist_n49/47(In47), LowerDist_n48/47(In47), LowerDist_n47/1(In1), LowerDist_n46/47(In47), LowerDist_n45/47(In47), LowerDist_n44/47(In47), LowerDist_n43/47(In47), LowerDist_n42/47(In47), LowerDist_n41/47(In47), LowerDist_n31/47(In47), LowerDist_n40/47(In47), LowerDist_n39/47(In47), LowerDist_n38/47(In47), LowerDist_n37/47(In47), LowerDist_n36/47(In47), LowerDist_n35/47(In47), LowerDist_n34/47(In47), LowerDist_n33/47(In47), LowerDist_n32/47(In47), LowerDist_n20/47(In47), LowerDist_n19/47(In47), LowerDist_n18/47(In47), LowerDist_n17/47(In47), LowerDist_n16/47(In47), LowerDist_n15/47(In47), LowerDist_n14/47(In47), LowerDist_n13/47(In47), LowerDist_n12/47(In47), LowerDist_n11/47(In47), LowerDist_n10/47(In47), LowerDist_n9/47(In47), LowerDist_n8/47(In47), LowerDist_n7/47(In47), LowerDist_n6/47(In47), LowerDist_n5/47(In47), LowerDist_n4/47(In47), LowerDist_n3/47(In47), LowerDist_n2/47(In47), LowerDist_n1/47(In47), Gateway Out39/1
  dist_k49/1 -> LowerDist_n10/49(In49), LowerDist_n9/49(In49), LowerDist_n8/49(In49), LowerDist_n7/49(In49), LowerDist_n6/49(In49), LowerDist_n5/49(In49), LowerDist_n4/49(In49), LowerDist_n3/49(In49), LowerDist_n2/49(In49), LowerDist_n1/49(In49), LowerDist_n49/1(In1), LowerDist_n48/49(In49), LowerDist_n47/49(In49), LowerDist_n46/49(In49), LowerDist_n45/49(In49), LowerDist_n44/49(In49), LowerDist_n43/49(In49), LowerDist_n42/49(In49), LowerDist_n41/49(In49), LowerDist_n31/49(In49), LowerDist_n40/49(In49), LowerDist_n39/49(In49), LowerDist_n38/49(In49), LowerDist_n37/49(In49), LowerDist_n36/49(In49), LowerDist_n35/49(In49), LowerDist_n34/49(In49), LowerDist_n33/49(In49), LowerDist_n32/49(In49), LowerDist_n30/49(In49), LowerDist_n29/49(In49), LowerDist_n28/49(In49), LowerDist_n27/49(In49), LowerDist_n26/49(In49), LowerDist_n25/49(In49), LowerDist_n24/49(In49), LowerDist_n23/49(In49), LowerDist_n22/49(In49), LowerDist_n21/49(In49), LowerDist_n20/49(In49), LowerDist_n19/49(In49), LowerDist_n18/49(In49), LowerDist_n17/49(In49), LowerDist_n16/49(In49), LowerDist_n15/49(In49), LowerDist_n14/49(In49), LowerDist_n13/49(In49), LowerDist_n12/49(In49), LowerDist_n11/49(In49), Gateway Out42/1
  dist_k1/1 -> LowerDist_n10/10(In10), LowerDist_n9/9(In9), LowerDist_n8/8(In8), LowerDist_n7/7(In7), LowerDist_n6/6(In6), LowerDist_n5/5(In5), LowerDist_n4/4(In4), LowerDist_n3/3(In3), LowerDist_n2/2(In2), LowerDist_n1/1(In1), LowerDist_n41/41(In41), LowerDist_n42/42(In42), LowerDist_n43/43(In43), LowerDist_n44/44(In44), LowerDist_n45/45(In45), LowerDist_n46/46(In46), LowerDist_n47/47(In47), LowerDist_n48/48(In48), LowerDist_n49/49(In49), LowerDist_n31/31(In31), LowerDist_n32/32(In32), LowerDist_n33/33(In33), LowerDist_n34/34(In34), LowerDist_n35/35(In35), LowerDist_n36/36(In36), LowerDist_n37/37(In37), LowerDist_n38/38(In38), LowerDist_n40/40(In40), LowerDist_n39/39(In39), LowerDist_n21/21(In21), LowerDist_n22/22(In22), LowerDist_n23/23(In23), LowerDist_n24/24(In24), LowerDist_n25/25(In25), LowerDist_n26/26(In26), LowerDist_n27/27(In27), LowerDist_n28/28(In28), LowerDist_n30/30(In30), LowerDist_n29/29(In29), LowerDist_n11/11(In11), LowerDist_n12/12(In12), LowerDist_n13/13(In13), LowerDist_n14/14(In14), LowerDist_n15/15(In15), LowerDist_n16/16(In16), LowerDist_n17/17(In17), LowerDist_n18/18(In18), LowerDist_n20/20(In20), LowerDist_n19/19(In19), Gateway Out/1
  Gateway Out28/1 -> Mux2/2
  Gateway Out27/1 -> Mux2/1
  Mux2/1 -> Display3/1
  Sum_wxWinning_n77/1 -> Sum_wxWinning_n87/2
  Sum_wxWinning_n78/1 -> Sum_wxWinning_n88/2
  Sum_wxWinning_n87/1 -> Gateway Out27/1, WinningNeuron_wx/1
  Sum_wxWinning_n88/1 -> Gateway Out28/1, WinningNeuron_wy/1
  Mux/1 -> Minimum/1, Sort/1, Display1/1
  Minimum/2 -> Display/1
  Minimum/1 -> Display2/1, To Workspace1/1
  Sort/1 -> Display54/1
  Sort/2 -> Display55/1, To Workspace/1
